simulink model "fangzhen"  (R2018a)
settings: Solver=FixedStepAuto  StartTime=0.0  StopTime=120  FixedStep=0.01  RelTol=1e-3
libraries: simulink x6
(part 1 of 2)
settings Model: Creator=WZJ  LastModifiedBy=Zijian
settings SolverCC: ZeroCrossAlgorithm=Adaptive
settings DebuggingCC: MaxConsecutiveZCsMsg=none

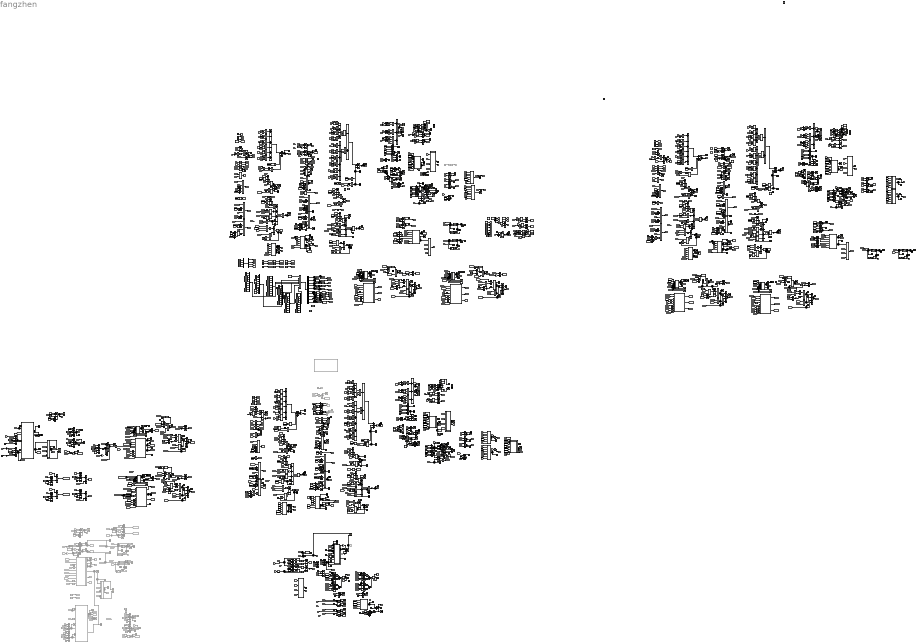
== system fangzhen ==
  note: 视野边界相撞
  note: 领导者机器人及其参数
  note: 相对坐标刚体队形
  note: 车辆模型
  note: 计算自变量
  note: 误差计算
  note: 切换初始位置k0
  note: 计算并选择过渡段,上界
  note: 误差模型1
  note: 控制器
  note: 选择过渡段
  note: theta i不等于theta id
  note: 控制器
  note: 计算接触斜率
  note: 角度界的计算
  note: 参数计算
  note: 计算过渡段
  note: 庄洁
  note: 后车角（此处theta和fai方向相反）
  note: 后车角误差
  note: 计算过渡段
  note: 计算自变量
  note: 误差模型1
  note: 后车角误差
  note: 选择过渡段
  note: 误差计算
  note: 控制器
  note: 角度界的计算
  note: 计算接触斜率
  note: theta i不等于theta id
  note: 计算接触斜率
  note: 选择过渡段
  note: 计算并选择过渡段,上界
  note: 控制器
  note: 庄洁
  note: 车辆模型
  note: 参数计算
  note: 切换初始位置k0
  note: 切换初始位置k0
  note: 计算过渡段
  note: 计算并选择过渡段,xia界
  note: 计算自变量
  note: 后车角（此处theta和fai方向相反）
  note: 误差计算
  note: theta i不等于theta id
  note: 参数计算
  note: 误差模型1
  note: 后车角（此处theta和fai方向相反）
  note: 控制器
  note: 控制器
  note: 车辆模型
  note: 庄洁
  note: 计算并选择过渡段,上界
  note: 计算并选择过渡段,xia界
  note: 计算自变量
  note: 计算接触斜率
  note: 计算过渡段
  note: 计算自变量
  note: 切换初始位置k0
  note: 计算接触斜率
  note: 后车角误差
  note: 选择过渡段
  note: 选择过渡段
  note: 切换初始位置k0
  note: 计算过渡段
  note: 选择过渡段
  note: 切换初始位置k0
  note: 计算接触斜率
  note: 计算过渡段
  note: 计算并选择过渡段,xia界
  note: 计算自变量
  note: 修正角（注意内部的正负）
  Abs{,1..5} (6 alike) : Abs
  Add{1,4,22,65,71,83,87,98..99,114,132..133,171,184,188,198..200} (18 alike) : Sum  Inputs=+--
  Add{10,13,15,17,21,23..24,28,34,36..40,43..46,50,52,55,59,62..63,69,73,76,85,95..96,101..102,104,106..107,109,113,115,117,120,122..123,129..130,134,136..139,143,147,149,153,160,162..163,166,168..169,173,176,186,195..196,225..227,233,236,240,263,267} (72 alike) : Sum  Inputs=+-
  Add{9,11..12,19,25,27,33,41,47,49,53,56..57,61,66,72,74,77..78,81,88..89,92,94,100,111,116,125,128,141,145,150,152,158,164,170,174,177..178,182,189..190,194,223,231,238,265,270} (48 alike) : Sum
  Add105 : Sum  Inputs=-+
  Add{2,16,35,51,108} (5 alike) : Sum  Inputs=+++
  Add{18,93,110,127,144,193,228,234} (8 alike) : Sum  Inputs=++-
  Add{20,112,146,175} (4 alike) : Sum  Inputs=+-+-
  Add{90..91,118,126,191..192} (6 alike) : Sum  Inputs=++--
  Add{119,135,140,224,230,264} (6 alike) : Sum  Inputs=++++
  Add{29,70,86,121,154,187} (6 alike) : Sum  Inputs=2
  Add{32,48,54,60,67..68,75,80,84,97,124,157,181,197} (14 alike) : Sum  Inputs=+-+
  Add14 : Sum  Inputs=-+
  Add{142,229,232,266} (4 alike) : Sum  Inputs=--
  Add148 : Sum  Inputs=+---
  Add{26,151,185,201,204..205,235,237,239} (9 alike) : Sum  Inputs=+-+--
  Add167 : Sum  Commented=on  Inputs=+--
  Add{172,207..208,210} (4 alike) : Sum  Commented=on  Inputs=+-+--
  Add{58,64,79,82,179,183} (6 alike) : Sum  Inputs=+++-
  Add180 : Sum  Commented=on  Inputs=+--
  Add211 : Sum  Commented=on  Inputs=+-+-
  Add212 : Sum  Commented=on  Inputs=+---
  Add213 : Sum  Commented=on  Inputs=+-+-
  Add214 : Sum  Commented=on  Inputs=+---
  Add42 : Sum  Inputs=-+
  Atan : Trigonometry  Operator=atan2
  Clock{2,5..6,8..11,24} (8 alike) : Clock
  Clock3 : Clock  Commented=on
  Clock4 : Clock  Commented=on
  Constant{1..3,49,54,56,69,72,79,98,118,124..125,138,147,161..162,175} (18 alike) : Constant  Value=3
  Constant{7,10,30,32,43,59,73,90,108,113,128,154,165..166,212,215,569..570,573} (19 alike) : Constant  Value=0.1
  Constant{8,23,25,28..29,31,33,35,46,48,53,64..66,70,74,84,87,91,94,100..102,109,111,117,123,134..135,140,145,151,156,160,171..172,177,192,213,264,289,293,543,564,568,572} (46 alike) : Constant
  Constant103 : Constant  Commented=on
  Constant{14,104..106,150,211,218} (7 alike) : Constant  Value=100
  Constant{4,62,85,93,107,132,157,169,214} (9 alike) : Constant  Value=0.01
  Constant{5,11,17,21..22,24,26..27,286..288} (11 alike) : Constant  Value=0.05
  Constant110 : Constant  Commented=on
  Constant{6,12..13,38..39,41,83,187,190,193..194} (11 alike) : Constant  Value=0
  Constant{18,50..51,57,67,82,89,95,120..121,126,149,153,155} (14 alike) : Constant  Value=pi*(87-7)/180
  Constant122 : Constant  Value=-0.3
  Constant127 : Constant  Value=1.5
  Constant{130,141,267,270,273,275,294,296,298} (9 alike) : Constant  Value=pi*87/180
  Constant133 : Constant  Value=0.2
  Constant{20,80..81,96..97,99,137,144,148,158..159,189,200..201,268..269,271,274,276,295,297,299,562} (23 alike) : Constant  Value=pi
  Constant143 : Constant  Value=pi*13/12
  Constant{9,15,78,86,92,565,567} (7 alike) : Constant  Value=10
  Constant152 : Constant  Value=0.3
  Constant{16,37,40,42} (4 alike) : Constant  Value=0.5
  Constant163 : Constant  Value=1.5
  Constant168 : Constant  Value=2
  Constant170 : Constant  Value=0.2
  Constant173 : Constant  Value=pi*13/12
  Constant{176,186,216,220} (4 alike) : Constant  Value=5
  Constant178 : Constant  Value=0.0001
  Constant182 : Constant  Value=50
  Constant185 : Constant  Value=20
  Constant19 : Constant  Value=-0.5
  Constant195 : Constant  Value=0.075
  Constant196 : Constant  Value=11.8  VectorParams1D=off
  Constant202 : Constant  Value=0.153  VectorParams1D=off
  Constant203 : Constant  Value=0.1  VectorParams1D=off
  Constant210 : Constant  Value=2
  Constant217 : Constant  Value=0.0001
  Constant219 : Constant  Value=20
  Constant243 : Constant  Value=-0.25
  Constant247 : Constant  Value=0.25
  Constant265 : Constant  Value=pi*11/12
  Constant36 : Constant  Value=6
  Constant{489,491,494,497,500,502} (6 alike) : Constant  Commented=on  Value=pi*87/180
  Constant490 : Constant  Commented=on  Value=-0.1
  Constant492 : Constant  Commented=on  Value=0.1
  Constant493 : Constant  Commented=on
  Constant{495..496,498,501,503} (5 alike) : Constant  Commented=on  Value=pi
  Constant499 : Constant  Commented=on  Value=-1
  Constant52 : Constant  Value=-0.3
  Constant{534,544,551,563} (4 alike) : Constant  Value=pi/2
  Constant538 : Constant  Value=1000
  Constant539 : Constant  Value=-0.5
  Constant545 : Constant  Value=pi*2
  Constant546 : Constant  Value=pi*3/2
  Constant547 : Constant  Commented=on  Value=pi/2
  Constant566 : Constant  Value=1000
  Constant63 : Constant  Value=0.2
  Constant68 : Constant  Value=0.15
  Constant71 : Constant  Value=0.15  VectorParams1D=off
  Constant75 : Constant  Commented=on  Value=2.828
  Constant76 : Constant  Commented=on  Value=pi*5/6
  Constant88 : Constant  Value=0.3
  Cos{1,3,7,11} (4 alike) : Trigonometry  Operator=cos
  Cos{2,4,8,12} (4 alike) : Trigonometry
  Demux : Demux  Outputs=10
  Demux1 : Demux
  Derivative{,1..45,47,50..58,61..64,66} (61 alike) : Derivative
  Divide{1..3,14..15,30,37,41,43,54..55,62} (12 alike) : Product
  Divide{5..6,9..11,21..22,25..27,35..36,38..40,42,45..46,49..51,60..61,63} (24 alike) : Product  Inputs=***
  Divide{7..8,12..13,23..24,28..29,47..48,52..53} (12 alike) : Product  Inputs=4
  Divide{16,18..19,31,33..34,56,58..59} (9 alike) : Product  Inputs=**
  Divide17 : Product  Inputs=3
  Divide20 : Product  Inputs=*/
  Divide32 : Product  Inputs=3
  Divide4 : Product  Inputs=*/
  Divide44 : Product  Inputs=*/
  Divide57 : Product  Inputs=3
  Foolower_1 : MATLAB Function  TreatAsAtomicUnit=on
  Foolower_2 : MATLAB Function  TreatAsAtomicUnit=on
  Foolower_3 : MATLAB Function  TreatAsAtomicUnit=on
  Foolower_4 : MATLAB Function  TreatAsAtomicUnit=on
  Foolower_5 : MATLAB Function  TreatAsAtomicUnit=on
  From1034 : From  Commented=on  GotoTag=xiajie_yuzhi_3
  From1046 : From  Commented=on  GotoTag=xi_pesai_3
  From1047 : From  Commented=on  GotoTag=xi_pesai_3_xia
  From{1087,1091,1093,1107..1108,1151} (6 alike) : From  Commented=on  GotoTag=pesai_d1_3
  From1088 : From  Commented=on  GotoTag=xi_pesai_0_xia_3
  From1089 : From  Commented=on  GotoTag=xi_shang
  From1090 : From  Commented=on  GotoTag=xi_xia
  From1092 : From  Commented=on  GotoTag=xi_pesai_0_3
  From1094 : From  Commented=on  GotoTag=pesai_d_a1_3
  From1095 : From  Commented=on  GotoTag=pesai_d_b1_3
  From{927,1097,1110,1148} (4 alike) : From  Commented=on  GotoTag=shang
  From{930,1098,1105,1113} (4 alike) : From  Commented=on  GotoTag=xia
  From1099 : From  Commented=on  GotoTag=xi_pesai_0_3
  From1100 : From  Commented=on  GotoTag=xi_pesai_0_xia_3
  From1101 : From  Commented=on  GotoTag=xi_pesai_0_3_qiehuan
  From1102 : From  Commented=on  GotoTag=xi_pesai_0_xia_3_qiehuan
  From1103 : From  Commented=on  GotoTag=xiajie_yuzhi_3
  From{1104,1109,1112,1147,1152} (5 alike) : From  Commented=on  GotoTag=fai_d_3
  From1106 : From  Commented=on  GotoTag=shangjie_yuzhi_3
  From1111 : From  Commented=on  GotoTag=pesai_d_3
  From1114 : From  Commented=on  GotoTag=pesai_d_3
  From1115 : From  Commented=on  GotoTag=pesai_d000
  From1118 : From  Commented=on  GotoTag=xi_shang
  From1119 : From  Commented=on  GotoTag=xi_xia
  From1143 : From  Commented=on  GotoTag=xi_pesai_3
  From1144 : From  Commented=on  GotoTag=xi_pesai_3_xia
  From1145 : From  Commented=on  GotoTag=shangjie_yuzhi_3
  From1146 : From  Commented=on  GotoTag=theta_id_3
  From1149 : From  Commented=on  GotoTag=ddd
  From1150 : From  Commented=on  GotoTag=theta_1
  From{934,1153..1155} (4 alike) : From  Commented=on  GotoTag=beta_3
  From932 : From  Commented=on  GotoTag=shang_
  From933 : From  Commented=on  GotoTag=xia_
  From935 : From  Commented=on  GotoTag=shangjie_yuzhi_3
  From938 : From  Commented=on  GotoTag=shang_
  From959 : From  Commented=on  GotoTag=xia_
  Gain{4,8..10,22..23,26,28,30,32,34,37,40,49,52,54,57,66,68..69,83..84,102} (23 alike) : Gain  Gain=-1
  Gain{13,24,41..44,71..72,75..76,100..101} (12 alike) : Gain  Gain=pi/2
  Gain{25,31,51,64..65,80,104,106..107} (9 alike) : Gain
  Gain{2..3,12,14..21,36,38..39,46..48,50} (18 alike) : Gain  Gain=0.5
  Gain{27,29,33,35,53,55} (6 alike) : Gain  Gain=3
  Gain{45,56,77..79} (5 alike) : Gain  Gain=-0.5
  Gain61 : Gain  Commented=on  Gain=-1
  Gain67 : Gain  Commented=on  Gain=-1
  Gain{81,86,91..92,95..96} (6 alike) : Gain  Commented=on  Gain=0.5
  Gain85 : Gain  Commented=on  Gain=-0.5
  Gain87 : Gain  Commented=on  Gain=-0.5
  Gain88 : Gain  Commented=on  Gain=-1
  Gain{89..90,93..94} (4 alike) : Gain  Commented=on
  Goto13 : Goto  Commented=on  GotoTag=l_d
  Goto19 : Goto  Commented=on  GotoTag=fai_d
  Goto243 : Goto  Commented=on  GotoTag=xi_pesai_3
  Goto263 : Goto  Commented=on  GotoTag=yipuxilong_pesai_3
  Goto290 : Goto  Commented=on  GotoTag=yipuxilong_pesai_3
  Goto325 : Goto  Commented=on  GotoTag=xi_pesai_3
  Goto368 : Goto  Commented=on  GotoTag=shang_
  Goto529 : Goto  Commented=on  GotoTag=xia_
  Goto534 : Goto  Commented=on  GotoTag=xi_pesai_0_xia_3_qiehuan
  Goto535 : Goto  Commented=on  GotoTag=xi_pesai_0_3_qiehuan
  Goto559 : Goto  Commented=on  GotoTag=yipuxilong_pesai_3
  Goto560 : Goto  Commented=on  GotoTag=pesai_d_b1_3
  Goto561 : Goto  Commented=on  GotoTag=pesai_d_a1_3
  Goto562 : Goto  Commented=on  GotoTag=beta_3
  Goto563 : Goto  Commented=on  GotoTag=xi_pesai_0_3
  Goto564 : Goto  Commented=on  GotoTag=xi_pesai_0_xia_3
  Goto565 : Goto  Commented=on  GotoTag=shangjie_yuzhi_3
  Goto566 : Goto  Commented=on  GotoTag=xiajie_yuzhi_3
  Goto567 : Goto  Commented=on  GotoTag=xi_pesai_3
  Goto568 : Goto  Commented=on  GotoTag=xi_pesai_3_xia
  Goto569 : Goto  Commented=on  GotoTag=ddd
  Goto570 : Goto  Commented=on  GotoTag=pesai_d_3
  Goto571 : Goto  Commented=on  GotoTag=pesai_d000
  Goto572 : Goto  Commented=on  GotoTag=xi_shang
  Goto573 : Goto  Commented=on  GotoTag=xi_xia
  Goto584 : Goto  Commented=on  GotoTag=C_3
  Integrator{5..8,10,15..18,20..22,24..29,34,39..44} (25 alike) : Integrator
  Integrator{9,11,30,45} (4 alike) : Integrator  InitialConditionSource=external
  Integrator12 : Integrator  InitialCondition=1.1
  Integrator13 : Integrator  InitialCondition=1
  Integrator14 : Integrator  InitialCondition=1.3
  Integrator19 : Integrator  InitialCondition=0.48236-0.1
  Integrator23 : Integrator  InitialCondition=-0.93185-0.5
  Integrator3 : Integrator  InitialCondition=0.8
  Integrator32 : Integrator  InitialCondition=0.8
  Integrator33 : Integrator  InitialCondition=-1
  Integrator35 : Integrator  InitialCondition=0.1
  Integrator36 : Integrator  InitialCondition=1.51763+0.1
  Integrator37 : Integrator  InitialCondition=-0.93185-0.5
  Integrator38 : Integrator  InitialCondition=1
  Integrator4 : Integrator  InitialCondition=0.1
  Integrator47 : Integrator  InitialCondition=-2.8637-0.5
  MATLAB Function : MATLAB Function  TreatAsAtomicUnit=on
  MATLAB Function1 : MATLAB Function  TreatAsAtomicUnit=on
  MATLAB Function10 : MATLAB Function  TreatAsAtomicUnit=on
  MATLAB Function13 : MATLAB Function  Commented=on  TreatAsAtomicUnit=on
  MATLAB Function14 : MATLAB Function  TreatAsAtomicUnit=on
  MATLAB Function15 : MATLAB Function  TreatAsAtomicUnit=on
  MATLAB Function16 : MATLAB Function  TreatAsAtomicUnit=on
  MATLAB Function17 : MATLAB Function  TreatAsAtomicUnit=on
  MATLAB Function2 : MATLAB Function  TreatAsAtomicUnit=on
  MATLAB Function20 : MATLAB Function  Commented=on  TreatAsAtomicUnit=on
  MATLAB Function22 : MATLAB Function  TreatAsAtomicUnit=on
  MATLAB Function23 : MATLAB Function  TreatAsAtomicUnit=on
  MATLAB Function25 : MATLAB Function  TreatAsAtomicUnit=on
  MATLAB Function26 : MATLAB Function  TreatAsAtomicUnit=on
  MATLAB Function27 : MATLAB Function  Commented=on  TreatAsAtomicUnit=on
  MATLAB Function29 : MATLAB Function  TreatAsAtomicUnit=on
  MATLAB Function3 : MATLAB Function  TreatAsAtomicUnit=on
  MATLAB Function30 : MATLAB Function  TreatAsAtomicUnit=on
  MATLAB Function32 : MATLAB Function  TreatAsAtomicUnit=on
  MATLAB Function36 : MATLAB Function  TreatAsAtomicUnit=on
  MATLAB Function37 : MATLAB Function  TreatAsAtomicUnit=on
  MATLAB Function38 : MATLAB Function  TreatAsAtomicUnit=on
  MATLAB Function39 : MATLAB Function  TreatAsAtomicUnit=on
  MATLAB Function4 : MATLAB Function  TreatAsAtomicUnit=on
  MATLAB Function47 : MATLAB Function  TreatAsAtomicUnit=on
  MATLAB Function48 : MATLAB Function  TreatAsAtomicUnit=on
  MATLAB Function49 : MATLAB Function  TreatAsAtomicUnit=on
  MATLAB Function50 : MATLAB Function  TreatAsAtomicUnit=on
  MATLAB Function52 : MATLAB Function  TreatAsAtomicUnit=on
  MATLAB Function7 : MATLAB Function  TreatAsAtomicUnit=on
  MATLAB Function8 : MATLAB Function  TreatAsAtomicUnit=on
  MATLAB 需要跑30s6 : MATLAB Function  TreatAsAtomicUnit=on
  Math Function{1..3,8..11,19..21,28,33,35,40..43,50} (18 alike) : Math  Operator=pow  SaturateOnIntegerOverflow=on
  Math Function{5..7,12..14,16..18,22..27,29..32,34,37..39,44..49,51} (30 alike) : Math  Operator=square  SaturateOnIntegerOverflow=on
  Math Function15 : Math  SaturateOnIntegerOverflow=on
  Math Function36 : Math  SaturateOnIntegerOverflow=on
  Math Function4 : Math  SaturateOnIntegerOverflow=on
  Memory{1..5,7..8,11..12,17,20..22,29..31,36..41} (22 alike) : Memory
  Memory{14..16,18..19,23..24} (7 alike) : Memory  Commented=on
  Multiport Switch : MultiPortSwitch
  Multiport Switch1 : MultiPortSwitch
  Multiport Switch2 : MultiPortSwitch
  Multiport Switch3 : MultiPortSwitch  Commented=on
  Multiport Switch4 : MultiPortSwitch  Inputs=6
  Mux{,1..3,6,15} (6 alike) : Mux  Inputs=10
  Mux7 : Mux
  Product{1,3,13..14,16,23,26,29..30,38,42,47,50,54,57,61,72,76,79..80,84..85,90..91,97,108,111..112,118,131,134,136,139,147,149,153,162,165..166,172..173,179} (42 alike) : Product  Inputs=**
  Product{5,10,12,17..18,21..22,24..25,28,33,37,39,45..46,52,56,58,62..63,65..66,74,82,87,89,94..95,98..100,103..107,109..110,113..116,119..125,127,130,133,138,140,144..145,148,150,154..155,157,160,168,170..171,180..184,186..195,197,202,205} (83 alike) : Product
  Product{19,32,34,40,101,141} (6 alike) : Product  Inputs=**/
  Product{20,48,51,59,71,75,102,151,161} (9 alike) : Product  Inputs=***/
  Product{6,11,27,35..36,43..44,55,64,67..68,73,77,126,128..129,132,142..143,156,158,163,196,198} (24 alike) : Product  Inputs=*/
  Product{96,117,178,185} (4 alike) : Product  Inputs=/*
  Product135 : Product  Commented=on  Inputs=/*
  Product137 : Product  Inputs=3
  Product{8,41,49,53,60,69..70,78,146,152,159,164} (12 alike) : Product  Inputs=**//
  Product15 : Product  Inputs=3
  Product167 : Product  Inputs=***
  Product169 : Product  Inputs=*/*
  Product31 : Product  Inputs=3
  Product81 : Product  Inputs=***
  Product83 : Product  Inputs=*/*
  Product86 : Product  Inputs=***
  Product88 : Product  Inputs=*/*
  Product93 : Product  Commented=on  Inputs=/*
  Saturation : Saturate  UpperLimit=0.04  LowerLimit=0
  Saturation Dynamic{,1..5} (6 alike) : simulink/Discontinuities/Saturation Dynamic  OutMin=[]  OutMax=[]  OutDataTypeStr=Inherit: Same as second input  OutDataType=fixdt(1, 16)  OutScaling=2^-10  DoSatur=off
  Saturation{1,3..4,9..11,16} (7 alike) : Saturate  UpperLimit=1  LowerLimit=-1
  Saturation12 : Saturate  UpperLimit=0.05  LowerLimit=0
  Saturation13 : Saturate  UpperLimit=0.05  LowerLimit=0
  Saturation{5,14..15,22..23,26} (6 alike) : Saturate  UpperLimit=0.1
  Saturation21 : Saturate  UpperLimit=0.05  LowerLimit=0
  Scope{1..30,32,34..35,37..40,42..48,50..80,82..84,86..88,90..115,117..127,129..135,137..166,168,170..173,175..201,203..219,221..222,224..228,230..236,238..242,244..245,247..248,250..257,259..265,267..269,271,273..282,284..286,290..297,299..301,306,310,312..316,318..320,322..323,325..328,339,345,347,349,368..371,378..387,389..393,401..404,408..420,423..424,428,469,472,475..476,478..486,490..495,504,506..508,514,516,518..519} (356 alike) : Scope
  Scope{36,41,81,85,89,116,167,169,202,220,223,266,270,283,289,311,321,324,348,421,427,488..489,505} (24 alike) : Scope  NumInputPorts=2
  Scope{31,49,128,229,388,405,477} (7 alike) : Scope  NumInputPorts=3
  Scope{237,243,246,336,350..353,358..362,364,367,372..376,422,426,430..436} (29 alike) : Scope  Commented=on
  Scope304 : Scope  Commented=on  NumInputPorts=3
  Scope{305,307..309,363,365..366,425,429} (9 alike) : Scope  Commented=on  NumInputPorts=2
  Sign : Signum
  Sign1 : Signum
  Sin{1,3,5..6,9..10} (6 alike) : Trigonometry  Operator=cos
  Square1 : Math  Operator=square  SaturateOnIntegerOverflow=on
  Square2 : Math  Operator=square  SaturateOnIntegerOverflow=on
  Square3 : Math  Operator=square  SaturateOnIntegerOverflow=on
  Subsystem1 : Subsystem
  Subsystem2 : Subsystem
  Subsystem3 : Subsystem
  Subsystem4 : Subsystem
  Subsystem5 : Subsystem
  Subtract1 : Sum  Inputs=++-
  Subtract{8..10,16,18,20,26..27,30,32,35,55..56,58..59,62..63,65..66} (19 alike) : Sum  Inputs=+-
  Subtract11 : Sum  Inputs=++-
  Subtract12 : Sum  Inputs=-+-+
  Subtract13 : Sum  Inputs=--+++-
  Subtract{4,14,24,31,33..34,36,60..61} (9 alike) : Sum  Inputs=-+
  Subtract15 : Sum  Inputs=++-+
  Subtract17 : Sum  Inputs=+-+-++
  Subtract{7,19,29,39..40,57,64,67..68} (9 alike) : Sum
  Subtract2 : Sum  Inputs=-+-+
  Subtract21 : Sum  Inputs=++-
  Subtract22 : Sum  Inputs=-+-+
  Subtract23 : Sum  Inputs=--+++-
  Subtract25 : Sum  Inputs=++-++
  Subtract28 : Sum  Inputs=+-+-++
  Subtract3 : Sum  Inputs=--+++-
  Subtract37 : Sum  Inputs=-++
  Subtract38 : Sum  Inputs=++-++
  Subtract5 : Sum  Inputs=+-+-++
  Subtract6 : Sum  Inputs=++-+
  Subtract71 : Sum  Inputs=+-+
  Subtract72 : Sum  Inputs=+-+
  Switch11 : Switch  Criteria=u2 > Threshold  Threshold=-0.5
  Switch12 : Switch  Criteria=u2 > Threshold  Threshold=0.5
  Switch{5,8..9,13} (4 alike) : Switch  Threshold=0.01
  Switch14 : Switch  Criteria=u2 > Threshold  Threshold=-0.5
  Switch17 : Switch  Commented=on  Criteria=u2 > Threshold  Threshold=0.1
  Switch18 : Switch  Commented=on  Threshold=0.00001
  Switch3 : Switch  Commented=on  Threshold=0.00001
  Switch4 : Switch  Commented=on  Criteria=u2 > Threshold  Threshold=-0.1
  Switch7 : Switch  Criteria=u2 > Threshold  Threshold=0.5
  To Workspace1 : ToWorkspace  VariableName=x0  SaveFormat=Structure  SampleTime=-1
  To Workspace11 : ToWorkspace  VariableName=x3  SaveFormat=Structure  SampleTime=-1
  To Workspace12 : ToWorkspace  VariableName=y3  SaveFormat=Structure  SampleTime=-1
  To Workspace2 : ToWorkspace  VariableName=y0  SaveFormat=Structure  SampleTime=-1
  To Workspace3 : ToWorkspace  VariableName=x2  SaveFormat=Structure  SampleTime=-1
  To Workspace6 : ToWorkspace  VariableName=x1  SaveFormat=Structure  SampleTime=-1
  To Workspace7 : ToWorkspace  VariableName=y1  SaveFormat=Structure  SampleTime=-1
  To Workspace8 : ToWorkspace  VariableName=y2  SaveFormat=Structure  SampleTime=-1
  Trigonometric Function{,1..2,5,8,11..12,15,18,24,26,28,30..34,36,42,44..49,51..52,55,58,61,67,69,71..74,82,89,94..96,98,100,103..104} (45 alike) : Trigonometry
  Trigonometric Function{3..4,6..7,9..10,13..14,16..17,19..23,25,27,29,35,37..41,43,50,53..54,56..57,59..60,62..66,68,87,90,92..93,97,99,105..106} (46 alike) : Trigonometry  Operator=cos
  Trigonometric Function88 : Trigonometry  Operator=atan2
  Trigonometric Function91 : Trigonometry  Operator=atan2
  tag scope: beta1=global
  wires:
  Constant264/1 -> [l_d_3], [l_d_2], [l_d]
  Product113/1 -> Add11/1
  Cos1/1 -> Product113/2
  [xL] -> Add11/2
  Product114/1 -> Add12/1
  Trigonometric Function29/1 -> Product116/1
  Constant265/1 -> [fai_d]
  Add11/1 -> [xLhead]
  [theta_L] -> Trigonometric Function29/1
  [theta_L] -> Cos1/1
  Integrator12/1 -> To Workspace2/1, [yL]  "yi"
  Integrator11/1 -> [theta_L]  "theta_i"
  [theta_L] -> Cos2/1
  Constant83/1 -> [oumiga_L_dot], [vL_dot]
  [theta_L] -> Trigonometric Function34/1
  Product115/1 -> Integrator12/1
  Cos2/1 -> Product114/2
  Constant143/1 -> [fai_d_2]
  Integrator13/1 -> To Workspace1/1, [xL]  "xi"
  Add102/1 -> [fai_d_3]
  Product116/1 -> Integrator13/1
  [oumiga_L] -> Integrator11/1
  [vL] -> Product116/2, Product115/1
  Trigonometric Function34/1 -> Product115/2
  [d] -> Product113/1
  Constant71/1 -> [h]
  [yL] -> Add12/2
  Add12/1 -> [yLhead]
  Constant68/1 -> [d]
  [d] -> Product114/1
  Add116/1 -> Scope250/1, [yF1head]
  [oumiga_1] -> Scope89/1
  Divide22/1 -> Subtract13/5
  Memory7/1 -> Switch13/1
  Constant2/1 -> Math Function1/2
  Constant20/1 -> Subtract15/4
  MATLAB Function/1(thetaid_0) -> Scope26/1, [theta_id_0]
  Math Function17/1 -> Product53/4
  Memory3/1 -> MATLAB Function2/6(d1b)
  [pesai_dot] -> Divide26/3
  Product72/1 -> Add80/2
  [u_21] -> Add86/1
  [pesai_d_b1] -> Multiport Switch/3
  Gain26/1 -> Scope113/1, [u_12]
  [pesai] -> Trigonometric Function13/1
  MATLAB Function3/1(V) -> [v1_dot_liju], Integrator6/1, Scope123/1
  Divide30/1 -> Subtract13/1
  Product103/1 -> Add108/1
  [h] -> MATLAB Function29/7(h)
  Divide26/1 -> Subtract5/3
  [e_pesai_dot] -> Product97/1
  Constant70/1 -> Add34/1
  [xi_pesai_0] -> MATLAB Function/1(x0)
  [vL] -> Divide38/1
  Constant62/1 -> [row_wuqiong]
  [yita_l] -> Add78/1
  [pesai_d1] -> Multiport Switch/4
  Add73/1 -> Product69/3
  Divide21/1 -> Subtract13/3
  Math Function16/1 -> Add125/2
  [pesai_d1] -> Scope49/1, MATLAB Function1/2(d1)
  Subtract11/1 -> Scope137/1, [gama_dot]
  [l] -> Divide20/2
  Math Function25/1 -> Add76/2
  Divide27/1 -> Subtract5/5
  [theta_id] -> MATLAB Function/3(thetaid)
  [yita_l] -> Product69/2
  [pesai_d1_00_a1] -> Memory3/1
  Saturation Dynamic/1 -> Product55/1
  Integrator6/1 -> [v1], Scope109/1
  Constant46/1 -> Add123/1
  [oumiga_id] -> Add97/3
  [fai] -> Trigonometric Function49/1
  [rou_0] -> Add122/1
  [xi_l] -> Product35/2
  [oumiga_1] -> Subtract16/2
  Saturation4/1 -> Product87/1
  Foolower_2/1(ldot) -> [l], Scope145/1
  [vL] -> MATLAB Function30/1(VL)
  [k_yita_pesai] -> Product8/1  "k_yita_pesai"
  Constant96/1 -> Add90/4
  [k_ke_xi_l] -> Product89/2  "k_ke_xi_l"
  Constant81/1 -> Add112/4
  [e_pesai_dot] -> Add83/1
  [xi_l] -> Product67/2
  Add81/1 -> Scope23/1, Product10/2
  Add37/1 -> Scope17/1, Product41/3
  [pesai] -> Trigonometric Function12/1
  [oumiga_L] -> Scope150/1, Add93/1
  Product37/1 -> Add88/2
  [fai] -> Trigonometric Function36/1
  [k_ke_xi_pesai] -> Product15/2  "k_ke_xi_pesai"
  Derivative28/1 -> [fai_dot], Scope85/2
  [oumiga_id] -> Add95/2
  [z_l] -> Math Function1/1
  Product11/1 -> Gain26/1
  Derivative36/1 -> [e_l_dot]
  Gain24/1 -> Add120/2
  [row_wuqiong] -> Add94/2
  Constant69/1 -> Math Function19/2
  [pesai_d1] -> Switch14/3
  Math Function19/1 -> Product89/1
  Subtract7/1 -> Scope120/1, [gama]
  [theta_L] -> Add1/2
  Product13/1 -> Scope155/1, Add82/1
  Clock10/1 -> Switch13/2
  Trigonometric Function37/1 -> Divide29/3
  [pesai_fin_a1] -> Scope16/1, Scope49/3, MATLAB Function1/4(fin)
  [c1_l] -> Product90/2
  [h] -> MATLAB Function30/7(h)
  [fai] -> Trigonometric Function39/1
  [yipuxilong_l_dot] -> Product71/1
  [theta_1] -> Add115/2
  [row_wuqiong] -> Add104/2
  [fai] -> Trigonometric Function37/1
  [k_tiaota_a1] -> Product107/1
  [yita_pesai] -> Math Function16/1
  Integrator18/1 -> [oumiga_1], Scope111/1
  [theta_L] -> Add67/2
  [v1] -> MATLAB Function29/2(Vi)
  Product47/1 -> Add83/2
  Gain2/1 -> Add1/3
  [e_pesai_dot] -> Add87/1
  Constant75/1 -> Goto13/1
  [z_l] -> Divide3/2
  Add113/1 -> Scope108/1
  [theta_id] -> Add67/1
  Product51/1 -> [c2_pesai]
  [shangjie_yuzhi] -> Add84/3
  [yLhead] -> Foolower_2/2(yl)
  [xi_pesai_x_a1] -> Product107/2
  Add99/1 -> Product84/1
  [fai_dot] -> Divide38/3
  Add100/1 -> [z_l]
  Divide24/1 -> Subtract13/6
  Derivative2/1 -> MATLAB Function2/4(d1_dotu)
  Gain15/1 -> Add84/2
  Product1/1 -> Add82/3
  [oumiga_L] -> MATLAB Function30/6(oumiga_L)
  Trigonometric Function12/1 -> Divide34/2
  [oumiga_1] -> Add97/2
  Divide29/1 -> Subtract5/6
  [shangjie_yuzhi] -> Add117/1
  [theta_1] -> Subsystem1/11(In11)
  MATLAB Function30/1(y) -> Scope381/1
  Add87/1 -> Product13/1
  [shangjie_yuzhi] -> MATLAB Function/6(shangjie_yuzhi)
  [shangjie_yuzhi] -> MATLAB Function2/2(shangjie_yuzhi)
  [pesai_d1] -> Derivative2/1
  [pesai_d1_dot_a1] -> Add120/1
  Add104/1 -> Product56/1
  Add123/1 -> Gain13/1
  [pesai] -> Trigonometric Function41/1
  [xF1head] -> Subsystem1/8(In8)
  Integrator14/1 -> [y1], To Workspace7/1  "yi"
  Product54/1 -> Add82/4
  [u_pesai_1] -> MATLAB Function3/6(u2)
  Add91/1 -> [pesai_d1], Scope87/1
  Switch13/1 -> Switch14/1
  [h] -> Divide35/1
  Add67/1 -> Scope70/1, [xi_pesai_0]
  MATLAB Function29/1(y) -> Scope380/1
  [oumiga_1] -> MATLAB Function29/5(oumiga_i)
  Integrator16/1 -> Subtract7/2
  [v1] -> MATLAB Function30/2(Vi)
  Product36/1 -> Scope161/1, [yita_pesai]
  [vL] -> MATLAB Function29/1(VL)
  Saturation5/1 -> Scope60/1
  [k_yita_pesai] -> Product41/1  "k_yita_pesai"
  [theta_id_0] -> Add75/1
  Add111/1 -> Scope257/1, [xF1head]
  [c_d_l] -> Product87/2  "自适应参数"
  Add117/1 -> Saturation Dynamic/2
  [l] -> MATLAB Function29/8(L)
  [k_c_l2] -> Product5/1  "k_c_l2"
  Add86/1 -> [u_l_1], Scope103/1
  [fai_dot] -> Divide29/4
  [xi_l] -> Derivative35/1
  Product41/1 -> Scope28/1, [ke_xi_pesai]
  [l_d] -> Product102/3
  [c1_pesai] -> Product34/1
  Trigonometric Function24/1 -> Product101/2
  [yita_l] -> Add50/2
  Gain13/1 -> Sin1/1
  [fai] -> MATLAB Function30/3(fai)
  Saturation3/1 -> Product33/1
  [pesai] -> MATLAB Function29/4(pesai)
  Product71/1 -> [c2_l]
  [rou_0] -> Gain24/1
  [ke_xi_l] -> Math Function18/1
  [theta_1] -> Subtract15/2
  [l] -> MATLAB Function3/3(l)
  [theta_L] -> Add91/1
  [oumiga_L] -> Add95/1
  [oumiga_L] -> Divide24/2
  [fai_d] -> Add110/1
  [d] -> Product101/3
  Product104/1 -> Add116/1
  [d] -> Product100/1
  [h] -> Divide24/1
  Gain21/1 -> Add114/3
  Add124/1 -> Gain22/1
  Subtract15/1 -> [fai], Scope71/1
  [oumiga_L_dot] -> Divide27/3
  Add112/1 -> Add105/1, Scope117/1
  Gain3/1 -> Add2/2
  Trigonometric Function25/1 -> Product102/2
  Constant63/1 -> [row_0]
  [yipuxilong_pesai] -> Add125/1
  Cos7/1 -> Product100/2
  [fai] -> MATLAB Function29/3(fai)
  [c3_l] -> Product91/1
  Math Function22/1 -> Add63/2
  Add96/1 -> [e_pesai], Scope92/1, Derivative1/1
  [pesai_d1_00_a1] -> Scope6/1, Add119/3
  [k_c_pesai] -> Product34/3  "k_c_pesai"
  [e_pesai] -> Product14/2
  Math Function26/1 -> Scope14/1, Product8/4
  [xi_pesai_0_xia] -> MATLAB Function/2(x0_xia)
  Switch5/1 -> Switch7/3
  [h] -> Divide29/1
  [c1_l] -> Divide3/1
  [xi_pesai_0] -> Scope53/1, Switch7/2
  [oumiga_L] -> Subtract11/2
  Math Function27/1 -> Product15/1
  Switch14/1 -> Scope68/1, Scope73/1, Memory7/1, Scope69/1
  [xiajie_yuzhi] -> Add2/3
  [oumiga_1] -> Add93/3, Scope165/1
  [pesai_d1_dot_a1] -> Memory5/1
  [pesai_d1] -> MATLAB Function2/5(d1_fnu)
  [pesai_d1] -> MATLAB Function2/3(d1u)
  MATLAB Function2/3(d1_fn) -> [pesai_fin_a1]
  [pesai_d_a1] -> Multiport Switch/2
  Multiport Switch/1 -> [pesai_d]
  [theta_L] -> Add2/1
  [oumiga_1] -> MATLAB Function30/5(oumiga_i)
  Product106/1 -> Scope4/1, Add119/1
  Constant57/1 -> Gain3/1
  [c1_pesai_dot] -> Product13/2
  Product6/1 -> [c3_pesai]
  Add83/1 -> Product42/1
  Add97/1 -> Scope38/1
  Product90/1 -> Scope10/1, Add100/1
  [k_ke_xi_l] -> Product86/2  "k_ke_xi_l"
  Product97/1 -> Add124/2, Scope115/1
  [oumiga_1] -> Divide35/3
  Product67/1 -> [yita_l]
  [e_l] -> Product91/2
  Product91/1 -> Add98/2
  [xLhead] -> Subsystem1/7(In7)
  [vL] -> Divide33/1
  Switch7/1 -> Scope45/1, Scope57/1, Memory11/1, Scope46/1
  [h] -> Divide28/1
  [v1] -> Divide34/1
  Gain27/1 -> Scope156/1, Add82/2
  Constant18/1 -> Gain20/1
  [yF1head] -> Subsystem1/5(In5)
  [fai_dot] -> Divide25/3
  Divide20/1 -> Scope132/1, Square2/1, [l_ni1]  "求逆"
  MATLAB Function1/2(a) -> Scope58/1
  [theta_1] -> Add107/2
  MATLAB Function/2(a) -> Scope7/1, Multiport Switch/1
  [oumiga_L] -> Divide29/2
  Cos8/1 -> Product104/2
  [xi_l] -> Product71/3
  [xi_pesai_0] -> MATLAB Function2/1(x0)
  Trigonometric Function44/1 -> Divide24/3
  [yita_pesai] -> Add81/1
  [c3_pesai] -> Product97/2
  Integrator8/1 -> [theta_id], Scope116/1, Scope42/1
  MATLAB Function2/1(d1) -> [pesai_d1_00_a1]
  Product33/1 -> Scope112/1, Add124/3
  [theta_L] -> Subtract15/3
  Gain14/1 -> Add67/3
  [k_c_pesai2] -> Product12/1
  Subtract13/1 -> Divide37/1
  [l_d] -> Subtract18/2
  Divide32/1 -> Subtract14/1
  [c2_pesai] -> Add87/3
  Derivative34/1 -> Scope157/1, [yipuxilong_pesai_dot]
  [e_pesai] -> Scope163/1, Product36/1
  Gain10/1 -> [u_21]
  [fai_d] -> Subtract8/2
  [l_ni2] -> Divide32/2
  [c3_l] -> Product72/2
  [h] -> Divide23/1
  [yipuxilong_l] -> Add77/1
  Product8/1 -> Scope160/1, [c1_pesai]
  [fai] -> Derivative28/1
  [oumiga_L] -> Product103/1
  Divide35/1 -> Subtract12/3
  [pesai] -> Subtract15/1
  Product89/1 -> Scope11/1, Add100/2
  [yita_pesai] -> Math Function22/1
  [pesai] -> MATLAB Function30/4(pesai)
  Add1/1 -> Scope25/1, [xi_pesai_0_xia]
  Add106/1 -> Trigonometric Function24/1
  [theta_L] -> Add75/2
  Constant97/1 -> Add91/4
  Add84/1 -> MATLAB Function/4(theta_shang_xiuzheng)
  Add88/1 -> [z_pesai]
  [ke_xi_pesai] -> Math Function27/1
  Constant50/1 -> Gain21/1
  [theta_1] -> Scope116/2
  [yipuxilong_l] -> Derivative17/1
  [e_pesai] -> Product47/2
  [theta_id_0] -> Add114/1
  Product98/1 -> Integrator14/1
  [yipuxilong_l] -> Add89/1
  [u_22] -> Add86/2
  [ke_xi_pesai_dot] -> Product15/3
  Math Function2/1 -> Scope8/1, Product1/2
  Derivative32/1 -> Scope51/1, [ke_xi_pesai_dot]
  [z_pesai] -> Divide1/2
  [c1_pesai] -> Derivative21/1
  Product73/1 -> Gain28/1
  Integrator27/1 -> Scope29/1
  Math Function15/1 -> Product56/2
  Derivative25/1 -> Scope85/1
  Add90/1 -> Scope169/2, Add96/1, Scope86/1
  [row_0] -> Add104/1
  [yipuxilong_pesai] -> Add81/2
  Math Function1/1 -> Scope9/1, Product3/2
  Divide31/1 -> Subtract5/1
  [v1] -> Product99/2, Product98/1
  [yita_pesai] -> Add37/2
  Integrator25/1 -> Math Function21/1, Scope20/1, [c_d_pesai]
  [xF1head] -> Subsystem1/3(In3)
  Product85/1 -> Add99/2
  [e_l_dot] -> Add99/1
  Product108/1 -> Scope15/1, Add79/4
  [theta_L] -> Add84/1
  Add77/1 -> Product71/4
  Divide23/1 -> Subtract13/4
  [xiajie_yuzhi] -> MATLAB Function/7(xiajie_yuzhi)
  Divide25/1 -> Subtract5/2
  Constant1/1 -> Math Function2/2
  Add50/1 -> Product66/1
  [e_l_dot] -> Product72/1
  [k_c_l] -> Product88/2  "k_c_l"
  Add49/1 -> Product41/4
  [theta_id] -> Add91/3
  [yita_pesai] -> Add49/1
  Product46/1 -> Math Function15/1
  [h] -> Divide27/1
  [yita_pesai] -> Product41/2
  Product100/1 -> Add111/1
  [h] -> MATLAB Function3/4(h)
  Subtract8/1 -> Scope83/1, Derivative25/1
  [theta_1] -> Add90/3
  Add23/1 -> Integrator25/1
  Subtract5/1 -> Add80/1
  [v1] -> Divide26/1
  [fai_dot] -> Divide24/4
  Divide28/1 -> Subtract5/4
  Memory11/1 -> Switch5/1
  [pesai_dot] -> Divide23/4
  Divide34/1 -> Subtract12/2
  Subtract12/1 -> Divide32/1
  [fai] -> Subtract7/1
  [yita_l] -> Add73/2
  [xi_pesai_x_a1] -> Product105/2
  Product56/1 -> Add94/1
  [u_12] -> Add121/2
  [c2_pesai] -> Add83/3
  Math Function24/1 -> Add89/2
  [theta_id] -> Add1/1
  [oumiga_1] -> Scope386/1, Integrator9/1
  [yF1head] -> Foolower_2/4(yf1head)
  Trigonometric Function38/1 -> Divide36/2
  [yita_l] -> Math Function24/1
  Add76/1 -> Product71/2
  Product88/1 -> Abs1/1
  Square2/1 -> [l_ni2], Scope126/1
  [yipuxilong_pesai] -> Scope18/1, Add66/1
  [yipuxilong_pesai_dot] -> Product51/1
  [e_l] -> Product85/2
  Divide3/1 -> Saturation4/1
  [k_yita_l] -> Product53/1  "k_yita_l"
  [c3_pesai] -> Product47/1
  Add121/1 -> [u_pesai_1], Scope65/1
  Product101/1 -> Add108/2
  Divide33/1 -> Subtract12/1
  MATLAB Function1/1(y) -> [pesai_d_a1], Derivative26/1, Scope47/1
  [theta_L] -> Add101/2
  [c1_l] -> Product88/3
  Product12/1 -> Add23/2
  Integrator15/1 -> [x1], To Workspace6/1  "xi"
  [vL_dot] -> Divide30/1
  [v1] -> Divide21/1
  [vL_dot] -> Divide31/1
  [pesai] -> Trigonometric Function42/1
  [fai_dot] -> Subtract11/1
  Gain29/1 -> Add79/2
  [yipuxilong_pesai] -> Derivative34/1
  Derivative35/1 -> [xi_l_dot]
  Product53/1 -> [c1_l]
  [ke_xi_pesai] -> Math Function28/1
  Math Function29/1 -> Add77/2
  Integrator9/1 -> Scope296/1, [theta_1]  "theta_i"
  [theta_1] -> Cos8/1
  [fai] -> Trigonometric Function40/1
  Sin1/1 -> Product106/2
  Gain28/1 -> Scope114/1, [u_22]
  [oumiga_1] -> Divide23/2
  [oumiga_1] -> Divide28/2
  Add85/1 -> Integrator26/1
  Trigonometric Function13/1 -> Divide35/2
  Product102/1 -> Add108/3
  [pesai_fin_a1] -> Memory8/1
  Add95/1 -> Add62/2, Integrator27/1
  Trigonometric Function35/1 -> Divide28/3
  Trigonometric Function41/1 -> Divide21/2
  [yita_l] -> Math Function25/1
  [z_l] -> Product108/1
  Product86/1 -> Gain29/1
  Product107/1 -> Scope5/1, Add119/2
  [c1_l] -> Derivative23/1
  [ke_xi_l_dot] -> ?
  Memory5/1 -> MATLAB Function2/7(d1_dotb)
  Constant48/1 -> Add37/1
  MATLAB Function3/2(W) -> Scope124/1, [oumiga_1_dot_liju], Integrator18/1
  [theta_1] -> Trigonometric Function14/1
  [c1_pesai] -> Product42/2
  Product14/1 -> Add87/2
  Add98/1 -> Product90/1
  [theta_id] -> Add112/2
  [xi_pesai] -> Scope162/1, Product36/2
  [gama] -> Add105/2
  [k_z_l] -> Product3/1
  [xi_pesai_dot] -> Product6/1
  [vL] -> Product101/1
  Integrator26/1 -> Math Function20/1, Scope80/1, [c_d_l]
  Constant54/1 -> Math Function20/2
  Add79/1 -> Product73/1
  [pesai] -> Scope169/1
  Trigonometric Function18/1 -> Product98/2
  Derivative30/1 -> [xi_pesai_dot]
  [theta_id] -> Add101/1
  [yipuxilong_l] -> Add74/2
  Gain22/1 -> [u_11], Scope24/1
  [pesai_dot] -> Divide21/3
  [e_l] -> Product67/1
  Add107/1 -> Scope144/1, [beta1]
  Constant76/1 -> Goto19/1
  [fai_d] -> Add112/3
  [e_l_dot] -> Add98/1
  [k_z_pesai] -> Product1/1
  Math Function21/1 -> Product12/2
  [z_pesai] -> Product54/1
  Add114/1 -> Product96/2, [xi_pesai_xia], Scope143/1
  [k_tiaota_a1] -> Product105/1
  [yita_l] -> Add76/1
  Math Function28/1 -> Product37/1
  Add80/1 -> Scope40/1, Gain10/1
  Add93/1 -> Add62/1, Scope166/1, Integrator5/1
  [theta_id] -> Add115/1
  [d] -> Product104/1
  [oumiga_L_dot] -> Divide22/3
  [xi_l_dot] -> Product35/1
  Integrator5/1 -> Scope43/1
  [xLhead] -> Subsystem1/2(In2)
  [rou_0] -> Product55/2
  [theta_L] -> Add114/2
  [xi_pesai] -> Derivative30/1
  [c1_l_dot] -> Product84/2
  Product69/1 -> [ke_xi_l]
  [k_ke_xi_pesai_dot] -> Product54/2
  [yita_l] -> Math Function29/1
  Product105/1 -> Add122/2
  MATLAB Function2/2(d1_dot) -> [pesai_d1_dot_a1]
  Divide1/1 -> Saturation3/1
  [theta_L] -> Add110/2
  Add119/1 -> [pesai_jie_a1], Scope48/1
  [xF1head] -> Foolower_2/3(xf1head)
  Add94/1 -> Scope110/1, Gain66/1, [xi_l]
  [pesai] -> Trigonometric Function35/1
  Product10/1 -> Math Function26/1
  Add62/1 -> Scope90/1
  Add2/1 -> MATLAB Function/5(theta_xia_xiuzheng)
  Divide38/1 -> Subtract13/2
  [x1] -> Add111/2
  [c3_l] -> Product85/1
  [oumiga_L] -> MATLAB Function29/6(oumiga_L)
  [theta_L] -> Add107/1
  Add89/1 -> Product53/2
  [theta_id] -> Add106/2
  Derivative17/1 -> [yipuxilong_l_dot]
  [pesai_jie_a1] -> Scope21/1, Scope49/2, MATLAB Function1/3(jie)
  Subtract14/1 -> Add124/1
  [c1_pesai] -> Divide1/1
  [ke_xi_l] -> Math Function19/1
  Derivative31/1 -> Scope32/1
  [fai] -> Add90/2
  [theta_L] -> Add112/1
  [d] -> Product102/4
  [theta_id] -> Add113/2
  Derivative23/1 -> [c1_l_dot]
  [u_11] -> Add121/1
  [oumiga_L] -> Product102/1
  [e_l] -> Derivative36/1
  [c2_l] -> Add99/3
  Derivative26/1 -> Saturation5/1
  [pesai_d1] -> Switch7/1
  [c2_l] -> Add98/3
  [y1] -> Add116/2
  Subtract18/1 -> Scope154/1, [e_l]
  Add120/1 -> [k_tiaota_a1]
  Trigonometric Function43/1 -> Divide22/2
  Constant49/1 -> Math Function28/2
  Trigonometric Function42/1 -> Divide23/3
  Constant59/1 -> [k_row]
  Add125/1 -> Product8/2
  [xi_pesai_x_a1] -> Add123/2
  [yita_l] -> Add74/1
  [xi_pesai] -> Product8/3
  [oumiga_1] -> Subtract11/3
  Trigonometric Function46/1 -> Divide30/2
  [h] -> Divide22/1
  Constant87/1 -> Divide20/1
  [xi_pesai_0] -> MATLAB Function1/1(x0)
  Gain4/1 -> Product46/2
  [ke_xi_pesai] -> Derivative32/1
  Divide36/1 -> Subtract12/4
  [fai_dot] -> Add93/2, Scope164/1
  [h] -> Divide36/1
  Trigonometric Function40/1 -> Divide38/2
  Trigonometric Function23/1 -> Product103/2
  Math Function23/1 -> Scope19/1, Add66/2
  [oumiga_L] -> Divide36/3
  [z_pesai] -> Math Function2/1
  [theta_1] -> Subsystem1/1(In1)
  Trigonometric Function19/1 -> MATLAB Function3/2(c)
  Add74/1 -> Product69/4
  [xi_pesai] -> Product51/3
  [k_ke_xi_pesai] -> Product37/2  "k_ke_xi_pesai"
  [pesai_dot] -> Divide28/4
  [c_d_pesai] -> Gain25/1  "自适应参数"
  [yLhead] -> Subsystem1/9(In9)
  [c3_pesai] -> Product14/1
  Gain20/1 -> Add75/3
  [fai] -> Trigonometric Function43/1
  [fai_d] -> Add91/2
  Add34/1 -> Scope22/1, Product10/1
  Constant53/1 -> Add73/1
  [theta_L] -> Add109/1
  [fai] -> Trigonometric Function38/1
  Add78/1 -> Product66/2
  [xLhead] -> Foolower_2/1(xl)
  Trigonometric Function39/1 -> Divide31/2
  Add101/1 -> Scope146/1
  Add66/1 -> Scope13/1, Product51/4
  [ke_xi_l] -> Derivative16/1
  [xi_pesai] -> Product6/2
  [fai] -> Trigonometric Function46/1
  Trigonometric Function49/1 -> Divide33/2
  [k_ke_xi_l_dot] -> Product108/2
  [theta_1] -> Trigonometric Function18/1
  [yita_pesai] -> Add34/2
  Trigonometric Function36/1 -> Divide27/2
  Product99/1 -> Integrator15/1
  Product55/1 -> Scope50/1, [xi_pesai_x_a1]
  Constant65/1 -> Add50/1
  Constant82/1 -> Gain14/1
  [l] -> Subtract18/1
  [fai_dot] -> Add97/1
  [yita_pesai] -> Add63/1
  Product42/1 -> Add88/1
  Add122/1 -> Product106/1
  [theta_1] -> Cos7/1
  [e_pesai] -> Derivative31/1
  Divide37/1 -> Subtract14/2
  [theta_id] -> Add110/3
  [xi_l] -> Product53/3
  [pesai] -> Trigonometric Function48/1
  Math Function18/1 -> Product86/1
  [xi_pesai_0_xia] -> Scope72/1, Switch14/2
  [z_l] -> Product88/1
  Add115/1 -> Scope119/1
  [pesai_d] -> Add96/2, Scope27/1
  [oumiga_L] -> Subtract16/1
  Trigonometric Function48/1 -> Divide26/2
  [theta_1] -> Subsystem1/6(In6)
  [yita_pesai] -> Math Function23/1
  [z_pesai] -> Product34/2
  Derivative1/1 -> [e_pesai_dot]
  Product3/1 -> Add79/3
  Constant64/1 -> [yipuxilong_l]
  Constant51/1 -> Gain2/1
  Add63/1 -> Product51/2
  Add109/1 -> Trigonometric Function23/1
  Subtract16/1 -> Integrator16/1
  Gain9/1 -> [yipuxilong_pesai], Scope147/1
  [theta_L] -> Add90/1
  [ke_xi_l_dot] -> Product86/3
  [yLhead] -> Subsystem1/4(In4)
  Add108/1 -> Scope89/2, [oumiga_id], Integrator8/1
  Constant56/1 -> Math Function21/2
  Add75/1 -> Product96/1, [xi_pesai], Scope125/1
  Product15/1 -> Gain27/1
  [pesai] -> Trigonometric Function19/1, Trigonometric Function11/1
  Add82/1 -> Product11/1
  [yF1head] -> Subsystem1/10(In10)
  Product35/1 -> [c3_l]
  Add105/1 -> Scope104/1
  Trigonometric Function47/1 -> Divide25/2
  Derivative21/1 -> [c1_pesai_dot]
  Constant89/1 -> Gain15/1
  [l_ni1] -> Divide37/2
  Memory8/1 -> MATLAB Function2/8(d1_fnb)
  [c1_pesai] -> Product11/2, Scope158/1
  Product66/1 -> Math Function17/1
  Clock2/1 -> Gain4/1
  [vL] -> Divide25/1
  Subsystem1/1(seita_i) -> Scope99/1
  Trigonometric Function14/1 -> Product99/1
  [theta_L] -> Add106/1
  Add110/1 -> Trigonometric Function25/1
  [yipuxilong_pesai] -> Add49/2
  Product96/1 -> Gain9/1
  Clock5/1 -> Switch5/2
  [k_yita_l] -> Product69/1  "k_yita_l"
  [fai] -> Subtract8/1
  [c1_l] -> Product73/2
  [theta_id] -> Add109/2
  Math Function20/1 -> Product5/2
  Product5/1 -> Add85/2
  Subsystem1/2(Out3) -> Scope159/1, Derivative33/1, [pesai]
  [theta_1] -> Add113/1
  [k_row] -> Product46/1
  [u_l_1] -> MATLAB Function3/5(u1)
  [fai] -> Trigonometric Function44/1
  Derivative16/1 -> [ke_xi_l_dot], Scope118/1
  [xi_pesai_0] -> Add117/2
  Trigonometric Function11/1 -> MATLAB Function3/1(s)
  [fai] -> Trigonometric Function47/1
  [l_dot] -> Divide32/3
  [yipuxilong_l] -> Add78/2
  Product84/1 -> Add79/1
  Product87/1 -> Add80/3
  [ke_xi_l_dot_2] -> ?
  [oumiga_L] -> Divide8/2
  [l_2] -> Divide4/2
  Product112/1 -> Add132/2
  [e_pesai_2] -> Scope141/1, Product44/1
  [d] -> Product19/3
  Trigonometric Function3/1 -> Divide39/2
  Add127/1 -> Add45/1, Scope153/1, Integrator22/1
  [yita_l_2] -> Add52/2
  [v2] -> Product120/2, Product119/1
  Gain43/1 -> Sin6/1
  [u_l_1_2] -> MATLAB Function10/5(u1)
  Constant28/1 -> Add143/1
  Divide10/1 -> Subtract17/3
  [xi_pesai_2] -> Product59/3
  [oumiga_2] -> Divide39/3
  [fai_2] -> Trigonometric Function15/1
  [pesai_d1_dot_a1_2] -> Add136/1
  Integrator20/1 -> Math Function10/1, Scope218/1, [c_d_l_2]
  Derivative13/1 -> Scope220/1
  Add71/1 -> Product29/1
  Cos3/1 -> Product18/2
  Product50/1 -> Add72/1
  MATLAB Function10/1(V) -> [v2_dot_liju], Integrator28/1, Scope94/1
  Subtract6/1 -> [fai_2], Scope214/1
  [e_l_dot_2] -> Product76/1
  [fai_dot_2] -> Divide9/3
  Derivative22/1 -> [xi_pesai_dot_2]
  Trigonometric Function16/1 -> Divide13/3
  Divide42/1 -> Subtract3/2
  Product81/1 -> Gain35/1
  Add46/1 -> Product59/2
  [xi_pesai_0_xia_2] -> Scope215/1, Switch11/2
  Product17/1 -> Math Function31/1
  Add126/1 -> [pesai_d1_2], Scope222/1
  [h] -> Divide6/1
  MATLAB Function7/1(thetaid_0) -> Scope179/1, [theta_id_0_2]
  [theta_L] -> Add54/2
  Gain36/1 -> Add35/2
  [pesai_dot_2] -> Divide10/3
  [u_22_2] -> Add70/2
  Derivative41/1 -> [xi_l_dot_2]
  [yita_pesai_2] -> Product49/2
  [yipuxilong_l_2] -> Add53/2
  Add55/1 -> Product75/2
  Trigonometric Function4/1 -> Product120/1
  [oumiga_2] -> Subtract1/3
  Add129/1 -> Add45/2, Integrator21/1
  Product26/1 -> Scope122/1, Add58/4
  Subsystem2/1(seita_i) -> Scope227/1
  [theta_2] -> Add118/3
  [h] -> MATLAB Function25/7(h)
  [xi_pesai_2] -> Product64/2
  [pesai_2] -> Trigonometric Function10/1
  [oumiga_2] -> Subtract9/2
  Math Function9/1 -> Scope217/1, Product16/2
  Add56/1 -> Product75/4
  [theta_id_2] -> Add48/1
  [h] -> MATLAB Function26/7(h)
  Math Function34/1 -> Add56/2
  [e_pesai_2] -> Product30/2
  Integrator10/1 -> [oumiga_2], Scope75/1
  [v2] -> MATLAB Function26/2(Vi)
  [c_d_l_2] -> Product82/2  "自适应参数"
  Add35/1 -> MATLAB Function7/5(theta_xia_xiuzheng)
  Math Function5/1 -> Add33/2
  [pesai_d1_2] -> MATLAB Function17/3(d1u)
  Divide9/1 -> Subtract17/2
  Constant151/1 -> Divide4/1
  Multiport Switch1/1 -> [pesai_d_2]
  [c1_l_2] -> Product83/3
  Derivative11/1 -> [c1_l_dot_2]
  [xiajie_yuzhi_2] -> MATLAB Function7/7(xiajie_yuzhi)
  [theta_id_0_2] -> Add22/1
  Derivative44/1 -> MATLAB Function17/4(d1_dotu)
  [shangjie_yuzhi_2] -> MATLAB Function15/2(shangjie_yuzhi)
  Product117/1 -> Gain40/1
  Gain41/1 -> Sin5/1
  Product19/1 -> Add16/2
  [pesai_2] -> Trigonometric Function26/1
  Trigonometric Function30/1 -> Divide15/2
  [oumiga_2] -> MATLAB Function25/5(oumiga_i)
  Divide16/1 -> Subtract17/1
  [yita_pesai_2] -> Add41/1
  Constant125/1 -> Math Function11/2
  [fai_dot_2] -> Divide13/4
  [e_pesai_2] -> Derivative37/1
  Trigonometric Function6/1 -> MATLAB Function10/2(c)
  [theta_L] -> Add4/2
  Switch12/1 -> Scope59/1, Scope185/1, Memory12/1, Scope172/1
  Gain23/1 -> [u_11_2], Scope177/1
  [vL_dot] -> Divide16/1
  Clock11/1 -> Gain37/1
  [theta_2] -> Add24/2
  Derivative5/1 -> [e_pesai_dot_2]
  [oumiga_L] -> Scope127/1, Add127/1
  [oumiga_L] -> MATLAB Function25/6(oumiga_L)
  Add33/1 -> Product78/2
  [h] -> Divide13/1
  [c3_l_2] -> Product80/1
  [pesai_d1_dot_b1_2] -> Add141/1
  [yipuxilong_pesai_2] -> Scope170/1, Add47/1
  [yipuxilong_pesai_dot_2] -> Product59/1
  MATLAB Function17/2(d1_dot) -> [pesai_d1_dot_b1_2]
  Clock9/1 -> Switch9/2
  [c2_l_2] -> Add132/3
  Math Function30/1 -> Add55/2
  Divide4/1 -> Scope100/1, Square1/1, [l_ni1_2]  "求逆"
  Divide7/1 -> Subtract3/4
  MATLAB Function15/3(d1_fn) -> [pesai_fin_a1_2]
  Constant148/1 -> Add20/4
  Trigonometric Function31/1 -> Divide9/2
  [pesai_2] -> MATLAB Function25/4(pesai)
  [vL_dot] -> Divide15/1
  [u_pesai_1_2] -> MATLAB Function10/6(u2)
  Subsystem2/2(Out3) -> Scope135/1, [pesai_2]
  Trigonometric Function9/1 -> Product20/2
  Add92/1 -> Product60/2
  [yipuxilong_l_2] -> Add56/1
  Memory20/1 -> MATLAB Function17/6(d1b)
  [fai_2] -> MATLAB Function25/3(fai)
  [theta_id_2] -> Add10/1
  Clock8/1 -> Switch8/2
  [c_d_pesai_2] -> Gain31/1  "自适应参数"
  Product22/1 -> Add25/1
  [xi_pesai_2] -> Derivative22/1
  Add118/1 -> Scope167/2, Add130/1, Scope221/1
  Trigonometric Function17/1 -> Divide40/2
  [z_pesai_2] -> Product40/2
  Saturation14/1 -> Scope149/1
  [xi_pesai_x_b1_2] -> Product124/2
  Memory2/1 -> MATLAB Function15/6(d1b)
  Add58/1 -> Product77/1
  [theta_L] -> Add20/1
  Derivative18/1 -> [fai_dot_2], Scope220/2
  [fai_2] -> Trigonometric Function30/1
  [c1_pesai_2] -> Derivative10/1
  [xi_pesai_0_2] -> Add134/2
  [k_c_l_2] -> Product83/2  "k_c_l"
  Add19/1 -> [xF2head]
  Constant121/1 -> Gain17/1
  [theta_L] -> Add15/1
  [v2] -> Divide19/1
  Cos4/1 -> Product22/2
  Math Function14/1 -> Add92/2
  [pesai_jie_b1_2] -> Scope31/2, MATLAB Function16/3(jie)
  [e_pesai_dot_2] -> Product118/1
  Add136/1 -> [k_tiaota_a1_2]
  [yita_pesai_2] -> Add39/2
  Constant135/1 -> Add43/1
  Divide40/1 -> Subtract2/4
  [v2] -> MATLAB Function25/2(Vi)
  [pesai_2] -> MATLAB Function26/4(pesai)
  MATLAB Function26/1(y) -> Scope277/1
  [l_2] -> MATLAB Function25/8(L)
  [vL] -> MATLAB Function25/1(VL)
  Product29/1 -> Scope130/1, Add64/1
  Add138/1 -> Gain41/1
  Product109/1 -> Scope67/1, Add9/2
  [pesai_d1_dot_a1_2] -> Memory4/1
  [xi_pesai_x_a1_2] -> Add138/2
  Memory21/1 -> MATLAB Function15/8(d1_fnb)
  Memory22/1 -> MATLAB Function17/7(d1_dotb)
  [k_z_pesai_2] -> Product16/1
  [pesai_d1_00_b1_2] -> Memory20/1
  Gain32/1 -> Scope77/1, [u_12_2]
  Math Function3/1 -> Scope224/1, Product38/2
  [pesai_d1_2] -> Scope229/1, MATLAB Function4/2(d1)
  [xi_pesai_0_xia_2] -> MATLAB Function7/2(x0_xia)
  MATLAB Function16/1(y) -> [pesai_d_b1_2], Derivative45/1, Scope2/1
  [k_tiaota_b1_2] -> Product124/1
  [xi_pesai_0_xia_2] -> MATLAB Function16/1(x0)
  [pesai_d1_2] -> MATLAB Function15/3(d1u)
  MATLAB Function15/1(d1) -> [pesai_d1_00_a1_2]
  Constant98/1 -> Math Function3/2
  [pesai_dot_2] -> Divide12/4
  [theta_L] -> Add22/2
  [pesai_fin_a1_2] -> Memory21/1
  [pesai_d1_2] -> Derivative44/1
  Gain42/1 -> Add136/2
  Add135/1 -> [pesai_jie_a1_2], Scope228/1
  [shangjie_yuzhi_2] -> Add134/1
  [fai_d_2] -> Add18/1
  [yipuxilong_pesai_2] -> Derivative40/1
  [xi_l_2] -> Product43/2
  [vL] -> Product19/1
  [k_tiaota_a1_2] -> Product123/1
  [pesai_d1_00_b1_2] -> Scope148/1, Add140/3
  Divide2/1 -> Saturation9/1
  Product39/1 -> Scope76/1, Add32/3
  [ke_xi_pesai_2] -> Math Function32/1
  [theta_L] -> Add118/1
  [theta_id_2] -> Add24/1
  Gain12/1 -> Add48/3
  [pesai_fin_b1_2] -> Memory1/1
  [theta_L] -> Add48/2
  Add45/1 -> Scope225/1
  [yita_pesai_2] -> Add40/2
  Constant140/1 -> Add39/1
  Product119/1 -> Integrator3/1
  [c3_l_2] -> Product76/2
  [pesai_dot_2] -> Divide7/4
  Divide41/1 -> Subtract4/2
  Constant124/1 -> Math Function10/2
  Trigonometric Function33/1 -> Divide18/2
  [oumiga_L] -> Subtract1/2
  [pesai_2] -> Trigonometric Function3/1
  [yita_pesai_2] -> Math Function13/1
  Constant120/1 -> Gain19/1
  [fai_2] -> Trigonometric Function28/1
  [oumiga_2] -> Divide7/2
  [yF2head] -> Foolower_1/4(yf1head)
  [row_wuqiong_2] -> Add128/2
  Divide15/1 -> Subtract3/1
  Math Function33/1 -> Product45/1
  Subtract4/1 -> Add32/1
  [theta_2] -> Subsystem2/11(In11)
  Product58/1 -> Add69/2
  Math Function31/1 -> Scope102/1, Product78/4
  Constant123/1 -> Add52/1
  [oumiga_id_2] -> Add129/2
  Subtract17/1 -> Add60/1
  [oumiga_L_dot] -> Divide6/3
  Trigonometric Function28/1 -> Divide8/3
  Add43/1 -> Product65/1
  Product59/1 -> [c2_pesai_2]
  [theta_L] -> Add10/2
  Product76/1 -> Add60/2
  Add21/1 -> Scope64/1
  Saturation15/1 -> Scope234/1
  [d] -> Product18/1
  [fai_d_2] -> Add126/2
  Trigonometric Function27/1 -> Divide6/2
  [k_c_pesai_2] -> Product40/3  "k_c_pesai"
  [row_0_2] -> Add13/1
  Product118/1 -> Add32/2, Scope79/1
  [theta_2] -> Trigonometric Function5/1
  [xi_pesai_x_a1_2] -> Product121/2
  [oumiga_L] -> Subtract9/1
  [xi_pesai_x_b1_2] -> Add143/2
  MATLAB Function10/2(W) -> Scope95/1, [oumiga_2_dot_liju], Integrator10/1
  [pesai_d1_2] -> Derivative27/1
  Constant138/1 -> Math Function8/2
  [z_pesai_2] -> Divide2/2
  Add133/1 -> Product79/1
  Constant158/1 -> Add118/4
  Product63/1 -> Add128/1
  Add24/1 -> Scope88/1
  [c1_pesai_2] -> Product40/1
  Subtract9/1 -> Integrator7/1
  [fai_dot_2] -> Subtract1/1
  Product52/1 -> Math Function4/1
  [xLhead] -> Subsystem2/2(In2)
  [yLhead] -> Foolower_1/2(yl)
  Divide17/1 -> Subtract4/1
  [e_pesai_dot_2] -> Add65/1
  [yita_l_2] -> Add43/2
  [u_12_2] -> Add29/2
  [fai_dot_2] -> Divide42/3
  Trigonometric Function22/1 -> Divide5/2
  [z_l_2] -> Math Function3/1
  [vL] -> MATLAB Function26/1(VL)
  Add60/1 -> Scope195/1, Gain8/1
  Math Function4/1 -> Product63/2
  [k_c_pesai2_2] -> Product28/1
  [oumiga_L] -> Divide13/2
  [xi_pesai_0_2] -> MATLAB Function7/1(x0)
  [c1_pesai_dot_2] -> Product29/2
  Add69/1 -> Integrator20/1
  [theta_id_2] -> Add15/2
  Divide18/1 -> Subtract2/1
  [pesai_dot_2] -> Divide5/3
  Product123/1 -> Scope230/1, Add135/2
  [pesai_2] -> Trigonometric Function2/1
  Constant23/1 -> Add138/1
  [v2] -> Divide5/1
  [c1_pesai_2] -> Product50/2
  [fai_2] -> Trigonometric Function21/1
  Trigonometric Function32/1 -> Divide10/2
  [oumiga_L] -> Product21/1
  Divide14/1 -> Saturation10/1
  Math Function6/1 -> Product60/4
  [z_l_2] -> Divide14/2
  Constant126/1 -> Gain36/1
  Divide12/1 -> Subtract17/4
  [pesai_d_a1_2] -> Multiport Switch1/2
  [yipuxilong_pesai_2] -> Add33/1
  [fai_2] -> MATLAB Function26/3(fai)
  [v2] -> Divide10/1
  Gain17/1 -> Add4/3
  [xi_l_2] -> Product75/3
  [pesai_2] -> Trigonometric Function6/1, Trigonometric Function1/1
  [l_d_2] -> Product20/3
  Math Function32/1 -> Product31/1
  [ke_xi_l_2] -> Math Function8/1
  Add10/1 -> Scope107/1
  [xF2head] -> Foolower_1/3(xf1head)
  [pesai_2] -> Scope167/1
  Product83/1 -> Abs2/1
  Product44/1 -> Scope139/1, [yita_pesai_2]
  Derivative38/1 -> Scope205/1, [ke_xi_pesai_dot_2]
  Product68/1 -> [yita_l_2]
  [l_2] -> Subtract10/1
  [fai_dot_2] -> Divide8/4
  Product60/1 -> [c1_l_2]
  Add130/1 -> [e_pesai_2], Scope226/1, Derivative5/1
  Gain35/1 -> Add58/2
  Integrator28/1 -> [v2], Scope66/1
  [theta_id_2] -> Add17/2
  Saturation10/1 -> Product82/1
  [c3_pesai_2] -> Product118/2
  Add128/1 -> Scope74/1, Gain68/1, [xi_l_2]
  Product43/1 -> [c3_l_2]
  [c3_pesai_2] -> Product57/1
  [e_l_2] -> Derivative42/1
  [yLhead] -> Subsystem2/4(In4)
  Product126/1 -> Scope231/1, [xi_pesai_x_a1_2]
  Divide19/1 -> Subtract2/2
  Divide39/1 -> Subtract2/3
  Product111/1 -> Scope61/1, Add9/1
  [theta_L] -> Add126/1
  [fai_2] -> Trigonometric Function33/1
  Add61/1 -> Scope176/1, Product17/2
  [yita_l_2] -> Product70/2
  Add29/1 -> [u_pesai_1_2], Scope209/1
  [xiajie_yuzhi_2] -> Add35/3
  [k_z_l_2] -> Product38/1
  [k_ke_xi_pesai_2] -> Product45/2  "k_ke_xi_pesai"
  Add64/1 -> Product27/1
  [pesai_d_b1_2] -> Multiport Switch1/3
  Constant117/1 -> Add40/1
  [xi_pesai_0_2] -> Scope183/1, Switch12/2
  [pesai_fin_a1_2] -> Scope229/3, MATLAB Function4/4(fin)
  Trigonometric Function2/1 -> Divide19/2
  Add65/1 -> Product50/1
  Add72/1 -> [z_pesai_2]
  [theta_L] -> Add35/1
  [d] -> Product22/1
  Integrator22/1 -> Scope198/1
  [fai_2] -> Add118/2
  [yita_pesai_2] -> Math Function12/1
  [theta_id_2] -> Add21/2
  Product64/1 -> [c3_pesai_2]
  Product30/1 -> Add71/2
  [xLhead] -> Foolower_1/1(xl)
  Product78/1 -> Scope138/1, [c1_pesai_2]
  [fai_2] -> Trigonometric Function17/1
  Add141/1 -> [k_tiaota_b1_2]
  Gain33/1 -> Scope131/1, Add64/2
  Product20/1 -> Add16/3
  [theta_2] -> Cos4/1
  Derivative37/1 -> Scope186/1
  [d] -> Product20/4
  Product77/1 -> Gain34/1
  Constant149/1 -> Gain12/1
  [xLhead] -> Subsystem2/7(In7)
  [xi_pesai_2] -> Scope140/1, Product44/2
  Add53/1 -> Product70/4
  [pesai_d1_2] -> Multiport Switch1/4
  Subtract1/1 -> Scope101/1
  [oumiga_2] -> Scope223/1
  [yipuxilong_l_2] -> Add92/1
  Integrator29/1 -> [theta_id_2], Scope81/1, Scope197/1
  Constant159/1 -> Add126/4
  [yF2head] -> Subsystem2/5(In5)
  Memory1/1 -> MATLAB Function17/8(d1_fnb)
  Divide11/1 -> Subtract17/5
  Trigonometric Function5/1 -> Product119/2
  [k_tiaota_b1_2] -> Product127/1
  [theta_2] -> Trigonometric Function4/1
  Add22/1 -> Product117/2, [xi_pesai_2_xia], Scope105/1
  [pesai_d1_dot_b1_2] -> Memory22/1
  [theta_id_2] -> MATLAB Function7/3(thetaid)
  [theta_2] -> Cos3/1
  Switch9/1 -> Switch11/1
  Product45/1 -> Add72/2
  Foolower_1/1(ldot) -> [l_2], Scope106/1
  [h] -> Divide39/1
  Math Function8/1 -> Product109/1
  Saturation9/1 -> Product39/1
  [vL] -> Divide9/1
  [theta_2] -> Subsystem2/1(In1)
  [c1_l_2] -> Derivative11/1
  Integrator7/1 -> Subtract19/2
  Add25/1 -> [yF2head]
  [c1_l_2] -> Product111/2
  [k_ke_xi_pesai_2] -> Product31/2  "k_ke_xi_pesai"
  Add52/1 -> Product70/3
  [z_l_2] -> Product83/1
  Product121/1 -> Add137/2
  [gama_2] -> Add14/2
  Product79/1 -> Add58/1
  Gain40/1 -> [yipuxilong_pesai_2], Scope121/1
  [ke_xi_l_2] -> Math Function7/1
  [yita_l_2] -> Add55/1
  Derivative42/1 -> [e_l_dot_2]
  [xi_pesai_0_xia_2] -> Add139/1
  Derivative6/1 -> [ke_xi_l_dot_2], Scope84/1
  Add68/1 -> MATLAB Function7/4(theta_shang_xiuzheng)
  [c1_l_2] -> Product77/2
  Subtract2/1 -> Divide17/1
  Product38/1 -> Add58/3
  MATLAB Function25/1(y) -> Scope276/1
  [yipuxilong_l_2] -> Add57/2
  [e_l_2] -> Product80/2
  Add17/1 -> Trigonometric Function7/1
  Add140/1 -> [pesai_jie_b1_2], Scope3/1
  [pesai_d1_2] -> Scope31/1, MATLAB Function16/2(d1)
  [h] -> Divide8/1
  Derivative40/1 -> Scope133/1, [yipuxilong_pesai_dot_2]
  Add32/1 -> Gain23/1
  [fai_2] -> Trigonometric Function20/1
  [e_l_dot_2] -> Add132/1
  [xF2head] -> Subsystem2/3(In3)
  Gain19/1 -> Add22/3
  [xi_pesai_2] -> Product78/3
  [fai_2] -> Derivative18/1
  [xi_l_2] -> Product68/2
  [h] -> Divide12/1
  [pesai_d1_2] -> MATLAB Function15/5(d1_fnu)
  [oumiga_2] -> MATLAB Function26/5(oumiga_i)
  [xi_pesai_x_a1_2] -> Product123/2
  [yF2head] -> Subsystem2/10(In10)
  Product28/1 -> Add36/2
  [yita_l_2] -> Math Function30/1
  [theta_2] -> Subtract6/2
  Add39/1 -> Scope175/1, Product17/1
  [yita_l_2] -> Add57/1
  Add47/1 -> Scope98/1, Product59/4
  [oumiga_L] -> MATLAB Function26/6(oumiga_L)
  [oumiga_2] -> Divide12/2
  [h] -> Divide40/1
  [z_pesai_2] -> Math Function9/1
  MATLAB Function4/1(y) -> [pesai_d_a1_2], Derivative29/1, Scope152/1
  Add137/1 -> Product122/1
  Gain37/1 -> Product52/2
  Constant128/1 -> [k_row_2]
  [xi_l_dot_2] -> Product43/1
  [c3_pesai_2] -> Product30/1
  Trigonometric Function21/1 -> Divide42/2
  Sin6/1 -> Product125/2
  [fai_2] -> Subtract19/1
  [c1_l_2] -> Divide14/1
  Product128/1 -> Scope54/1, [xi_pesai_x_b1_2]
  [fai_2] -> Trigonometric Function27/1
  [yipuxilong_l_dot_2] -> Product75/1
  [pesai_fin_b1_2] -> Scope31/3, MATLAB Function16/4(fin)
  [rou_0_2] -> Gain42/1, Add137/1, Product126/2
  [theta_id_0_2] -> Add54/1
  [oumiga_2] -> Scope385/1, Integrator30/1
  [u_21_2] -> Add70/1
  Divide5/1 -> Subtract3/3
  Product16/1 -> Add64/3
  [theta_id_2] -> Add20/2
  [c1_l_dot_2] -> Product79/2
  Trigonometric Function15/1 -> Divide11/2
  Add14/1 -> Scope63/1
  [e_pesai_dot_2] -> Add71/1
  Product127/1 -> Scope52/1, Add140/2
  Constant132/1 -> [row_wuqiong_2]
  [k_tiaota_a1_2] -> Product121/1
  Add15/1 -> Trigonometric Function8/1
  [oumiga_L] -> Divide40/3
  Add9/1 -> [z_l_2]
  Add20/1 -> Add14/1, Scope82/1
  [fai_dot_2] -> Add127/2, Scope142/1
  [theta_L] -> Add18/2
  [k_yita_l_2] -> Product70/1  "k_yita_l"
  [l_d_2] -> Subtract10/2
  Constant133/1 -> [row_0_2]
  [k_yita_l_2] -> Product60/1  "k_yita_l"
  [theta_id_2] -> Add4/1
  Subtract20/1 -> Scope219/1, Derivative13/1
  [k_yita_pesai_2] -> Product49/1  "k_yita_pesai"
  [h] -> Divide7/1
  [pesai_d1_2] -> MATLAB Function17/5(d1_fnu)
  [pesai_d1_00_a1_2] -> Memory2/1
  [pesai_d_2] -> Add130/2, Scope180/1
  [yipuxilong_pesai_2] -> Add41/2
  Gain34/1 -> Scope78/1, [u_22_2]
  Add142/1 -> Product125/1
  [ke_xi_pesai_2] -> Math Function33/1
  [vL] -> Divide18/1
  [k_ke_xi_pesai_dot_2] -> Product61/2
  Product40/1 -> Abs3/1
  Derivative10/1 -> [c1_pesai_dot_2]
  Derivative27/1 -> MATLAB Function15/4(d1_dotu)
  Constant134/1 -> [yipuxilong_l_2]
  Add143/1 -> Gain43/1
  [yLhead] -> Subsystem2/9(In9)
  Add132/1 -> Product111/1
  Memory17/1 -> Switch9/1
  Constant118/1 -> Math Function33/2
  [yita_pesai_2] -> Add46/1
  [yita_pesai_2] -> Math Function5/1
  [ke_xi_pesai_dot_2] -> Product31/3
  [xi_pesai_x_b1_2] -> Product127/2
  [k_c_l2_2] -> Product58/1  "k_c_l2"
  [shangjie_yuzhi_2] -> Add68/3
  Add70/1 -> [u_l_1_2], Scope62/1
  [k_ke_xi_l_2] -> Product109/2  "k_ke_xi_l"
  Product120/1 -> Integrator4/1
  [c2_l_2] -> Add133/3
  Product31/1 -> Gain33/1
  [z_pesai_2] -> Product61/1
  [yipuxilong_pesai_2] -> Add61/2
  Subtract3/1 -> Divide41/1
  [theta_id_2] -> Add18/3
  Product80/1 -> Add133/2
  Add13/1 -> Product63/1
  [pesai_jie_a1_2] -> Scope229/2, MATLAB Function4/3(jie)
  Product125/1 -> Scope1/1, Add140/1
  Product57/1 -> Add65/2
  Add16/1 -> Scope223/2, [oumiga_id_2], Integrator29/1
  [xi_l_2] -> Product60/3
  Gain8/1 -> [u_21_2]
  Product61/1 -> Add64/4
  MATLAB Function7/2(a) -> Scope212/1, Multiport Switch1/1
  Integrator4/1 -> To Workspace3/1, Scope382/1, [x2]  "xi"
  [yita_l_2] -> Math Function14/1
  [ke_xi_pesai_2] -> Derivative38/1
  [c2_pesai_2] -> Add71/3
  [yipuxilong_l_2] -> Derivative7/1
  [pesai_2] -> Subtract6/1
  Derivative45/1 -> Saturation14/1
  Switch8/1 -> Switch12/3
  Math Function10/1 -> Product58/2
  Switch11/1 -> Scope210/1, Scope216/1, Memory17/1, Scope211/1
  [shangjie_yuzhi_2] -> MATLAB Function7/6(shangjie_yuzhi)
  Constant153/1 -> Gain16/1
  Memory4/1 -> MATLAB Function15/7(d1_dotb)
  [l_ni2_2] -> Divide17/2
  [oumiga_L] -> Add129/1
  Integrator21/1 -> Scope182/1
  [pesai_d1_2] -> Switch11/3
  [oumiga_L_dot] -> Divide11/3
  Trigonometric Function8/1 -> Product19/2
  [yita_l_2] -> Math Function34/1
  [c2_pesai_2] -> Add65/3
  Add18/1 -> Trigonometric Function9/1
  [ke_xi_l_2] -> Derivative6/1
  [e_pesai_2] -> Product57/2
  Trigonometric Function7/1 -> Product21/2
  [xiajie_yuzhi_2] -> MATLAB Function17/2(xiajie_yuzhi)
  Trigonometric Function10/1 -> Divide12/3
  [c3_l_2] -> Product112/1
  Gain18/1 -> Add54/3
  Divide8/1 -> Subtract3/6
  [fai_2] -> Trigonometric Function16/1
  [k_ke_xi_l_dot_2] -> Product26/2
  Divide6/1 -> Subtract3/5
  [theta_L] -> Subtract6/3
  [fai_2] -> Subtract20/1
  [pesai_d1_2] -> Switch12/1
  Add57/1 -> Product65/2
  Product65/1 -> Math Function6/1
  [ke_xi_l_dot_2] -> Product81/3
  [xi_pesai_0_2] -> MATLAB Function4/1(x0)
  [e_l_dot_2] -> Add133/1
  Add36/1 -> Integrator17/1
  [l_ni1_2] -> Divide41/2
  [vL] -> Divide42/1
  [oumiga_L] -> Product20/1
  Add4/1 -> Scope178/1, [xi_pesai_0_xia_2]
  MATLAB Function4/2(a) -> Scope232/1
  [yita_l_2] -> Add53/1
  Derivative7/1 -> [yipuxilong_l_dot_2]
  [xi_pesai_dot_2] -> Product64/1
  [h] -> MATLAB Function10/4(h)
  [row_wuqiong_2] -> Add13/2
  [xi_l_2] -> Derivative41/1
  [rou_0_2] -> Gain44/1, Product128/2, Add142/1
  Product82/1 -> Add60/3
  Product70/1 -> [ke_xi_l_2]
  [fai_d_2] -> Subtract20/2
  [e_l_2] -> Product68/1
  MATLAB Function16/2(a) -> Scope55/1
  MATLAB Function17/3(d1_fn) -> [pesai_fin_b1_2]
  [c1_pesai_2] -> Divide2/1
  Math Function13/1 -> Scope171/1, Add47/2
  Math Function11/1 -> Product28/2
  [h] -> Divide11/1
  Add40/1 -> Scope168/1, Product49/3
  Add48/1 -> Scope213/1, [xi_pesai_0_2]
  [u_11_2] -> Add29/1
  Add54/1 -> Product117/1, [xi_pesai_2], Scope96/1
  [k_ke_xi_l_2] -> Product81/2  "k_ke_xi_l"
  [x2] -> Add19/2
  Constant95/1 -> Gain18/1
  Integrator3/1 -> To Workspace8/1, Scope383/1, [y2]  "yi"
  [pesai_2] -> Trigonometric Function22/1
  Divide13/1 -> Subtract17/6
  [fai_2] -> Trigonometric Function31/1
  Square1/1 -> [l_ni2_2], Scope97/1
  [c1_pesai_2] -> Product27/2, Scope134/1
  [theta_2] -> Add21/1
  [theta_2] -> Scope81/2
  Product21/1 -> Add16/1
  Math Function12/1 -> Add46/2
  Gain16/1 -> Add68/2
  [k_yita_pesai_2] -> Product78/1  "k_yita_pesai"
  [xi_pesai_0_xia_2] -> MATLAB Function17/1(x0)
  [e_l_2] -> Product112/2
  [theta_L] -> Add68/1
  [z_l_2] -> Product26/1
  [theta_L] -> Add17/1
  [theta_2] -> Subsystem2/6(In6)
  Sin5/1 -> Product122/2
  Trigonometric Function26/1 -> Divide7/3
  Derivative29/1 -> Saturation15/1
  Constant72/1 -> Math Function9/2
  [theta_id_2] -> Add126/3
  Subtract19/1 -> Scope93/1, [gama_2]
  Product18/1 -> Add19/1
  [pesai_d1_00_a1_2] -> Scope233/1, Add135/3
  [yita_pesai_2] -> Add61/1
  [oumiga_2] -> Add127/3, Scope151/1
  Product75/1 -> [c2_l_2]
  Integrator30/1 -> Scope384/1, [theta_2]  "theta_i"
  Integrator17/1 -> Math Function11/1, Scope173/1, [c_d_pesai_2]
  [xiajie_yuzhi_2] -> Add139/2
  [y2] -> Add25/2
  [xi_pesai_0_2] -> MATLAB Function15/1(x0)
  Gain31/1 -> Product39/2
  Trigonometric Function1/1 -> MATLAB Function10/1(s)
  Add41/1 -> Product49/4
  [pesai_2] -> Trigonometric Function32/1
  Memory12/1 -> Switch8/1
  Subtract10/1 -> Scope129/1, [e_l_2]
  [xF2head] -> Subsystem2/8(In8)
  Product124/1 -> Add142/2
  [fai_d_2] -> Add20/3
  Gain44/1 -> Add141/2
  Product122/1 -> Scope56/1, Add135/1
  Constant99/1 -> Subtract6/4
  Math Function7/1 -> Product81/1
  MATLAB Function15/2(d1_dot) -> [pesai_d1_dot_a1_2]
  Product27/1 -> Gain32/1
  Trigonometric Function20/1 -> Divide16/2
  [l_dot_2] -> Divide17/3
  MATLAB Function17/1(d1) -> [pesai_d1_00_b1_2]
  Product49/1 -> Scope181/1, [ke_xi_pesai_2]
  [l_2] -> MATLAB Function10/3(l)
  [k_row_2] -> Product52/1
  [ke_xi_l_dot_3] -> ?
  [xiajie_yuzhi_3] -> ?
  ? -> ?
  [shang_] -> ?
  Trigonometric Function74/1 -> Divide58/2
  Divide43/1 -> Saturation11/1
  [e_pesai_dot_3] -> Add188/1
  Constant130/1 -> Gain38/1
  [pesai_d_b1_3] -> Scope348/1, Multiport Switch2/3
  [ke_xi_l_3] -> Derivative12/1
  Product131/1 -> Scope247/1, Add179/4
  Constant79/1 -> Math Function35/2
  Subtract23/1 -> Divide62/1
  [yipuxilong_pesai_dot_3] -> Product151/1
  [fai_3] -> Trigonometric Function62/1
  [fai_3] -> MATLAB Function22/3(fai)
  [d] -> Product48/4
  Integrator42/1 -> Scope297/1
  Saturation11/1 -> Product140/1
  Add190/1 -> Scope371/1, Product152/2
  Product155/1 -> Add194/1
  MATLAB Function14/2(W) -> Scope236/1, [oumiga_3_dot_liju], Integrator35/1
  Add27/1 -> [z_l_3]
  [xia] -> Add239/4
  Gain79/1 -> Add239/3
  Divide61/1 -> Subtract22/4
  [xi_pesai_x_b1_3] -> Product197/2
  Product191/1 -> Add226/2
  [h] -> Divide53/1
  Gain54/1 -> Scope200/1, [u_22_3]
  [oumiga_3] -> Divide60/3
  [xi_pesai_3] -> Product185/1
  [oumiga_3] -> MATLAB Function22/5(oumiga_i)
  Trigonometric Function65/1 -> Divide63/2
  [xiajie_yuzhi_3] -> MATLAB Function37/5(xiajie_yuzhi)
  Gain51/1 -> Product140/2
  [c3_pesai_3] -> Product179/2
  [xi_l_3] -> Product161/3
  [theta_3] -> Subtract25/2
  [fai_d_3] -> Add235/1
  [pesai_fin_b1_3] -> Scope388/3, MATLAB Function37/4(fin)
  [theta_1] -> Add191/1
  [pesai_d_a1_3] -> Multiport Switch2/2
  [xF3head] -> Subsystem5/8(In8)
  [fai_3] -> Trigonometric Function74/1
  Product157/1 -> Math Function38/1
  Divide55/1 -> Subtract23/1
  Add153/1 -> [xi_pesai_0_shang_3_qiehuan]
  [xi_pesai_x_b1_3] -> Product194/2
  Product140/1 -> Scope196/1, Add157/3
  Derivative8/1 -> MATLAB Function38/4(d1_dotu)
  Subsystem5/2(Out3) -> [xia], Scope423/1, [pesai_4]
  [oumiga_1] -> Divide48/2
  [c1_l_3] -> Divide54/1
  [h] -> MATLAB Function22/7(h)
  Add26/1 -> Add153/2
  [pesai_d1_3] -> Add153/1
  [c1_l_3] -> Product163/2
  Constant141/1 -> Gain50/1
  Constant137/1 -> Add26/5
  [pesai_d1_00_a1_3] -> Scope411/1, Add224/3
  [k_c_pesai2_3] -> Product133/1
  [yF1head] -> Subsystem3/4(In4)
  [c3_l_3] -> Product173/1
  MATLAB Function38/1(d1) -> Scope413/1, [pesai_d1_00_b1_3]
  [yipuxilong_pesai_3] -> Add158/1
  Add225/1 -> [k_tiaota_a1_3]
  [h] -> Divide47/1
  [pesai_dot_3] -> Scope421/2
  Derivative43/1 -> [c1_l_dot_3]
  [theta_3] -> Add191/3
  Divide45/1 -> Subtract23/3
  [xia] -> Add235/4
  [xi_pesai_3] -> Scope261/1, Product143/2
  [x3] -> Add145/2
  Math Function37/1 -> Add158/2
  [yF3head] -> Subsystem5/5(In5)
  Divide44/1 -> Scope240/1, Square3/1, [l_ni1_3]  "求逆"
  [xF2head] -> Subsystem5/7(In7)
  Subsystem5/1(seita_i) -> Scope424/1
  [yF2head] -> Subsystem5/4(In4)
  MATLAB Function37/2(a) -> Scope391/1
  Derivative64/1 -> MATLAB Function36/4(d1_dotu)
  [xF2head] -> Subsystem5/2(In2)
  [yF3head] -> Subsystem5/10(In10)
  [d] -> Product74/1
  [pesai_3] -> Trigonometric Function52/1
  [fai_d_3] -> Add151/1
  Constant298/1 -> Gain79/1
  MATLAB Function38/2(d1_dot) -> Scope414/1, [pesai_d1_dot_b1_3]
  [v3] -> Product181/2, Product180/1
  [fai_d_3] -> Add239/1
  Product150/1 -> Add186/2
  Product194/1 -> Add232/2
  [pesai_jie_b1_3] -> Scope388/2, MATLAB Function37/3(jie)
  Constant297/1 -> Add237/5
  Add237/1 -> Add238/1
  Product62/1 -> Add51/1
  [pesai_d1_3] -> Add200/2
  Constant268/1 -> Add200/3
  [pesai_d1_3] -> Add236/1
  [fai_dot_3] -> Subtract21/1
  Add238/1 -> [pesai_d_b1_3]
  Gain38/1 -> Add26/3
  [xF3head] -> Foolower_3/3(xf1head)
  Add144/1 -> Trigonometric Function59/1
  Constant295/1 -> Add235/5
  [yita_l_3] -> Math Function46/1
  [rou_0_3] -> Add232/1
  [shangjie_yuzhi_3] -> Add223/1
  [oumiga_1] -> Divide61/3
  [theta_id_3] -> Add171/1
  Constant294/1 -> Gain77/1
  [xiajie_yuzhi_3] -> MATLAB Function38/2(xiajie_yuzhi)
  [theta_1] -> Add171/2
  Product137/1 -> Gain53/1
  Gain77/1 -> Add235/3
  [k_tiaota_a1_3] -> Product193/1
  [xF3head] -> Subsystem5/3(In3)
  Constant273/1 -> Gain46/1
  [theta_1] -> Add192/1
  Derivative61/1 -> Saturation23/1
  [pesai_d_a1_3000] -> Add152/2
  [xi_pesai_x_b1_3] -> Add233/2
  Foolower_3/1(ldot) -> [l_3], Scope244/1
  Add193/1 -> Add168/1, Scope265/1, Integrator42/1
  Gain75/1 -> Sin10/1
  Gain71/1 -> Sin9/1
  [xi_pesai_0_shang_3_qiehuan] -> MATLAB Function36/1(x0)
  MATLAB Function36/1(d1) -> [pesai_d1_00_a1_3]
  Product197/1 -> Scope389/1, Add230/2
  Product198/1 -> Scope390/1, [xi_pesai_x_b1_3]
  Constant275/1 -> Gain56/1
  Gain76/1 -> Add231/2
  Product180/1 -> Integrator32/1
  [y3] -> Add150/2
  [oumiga_3] -> MATLAB Function23/5(oumiga_i)
  [xia] -> Add237/4
  [k_tiaota_b1_3] -> Product197/1
  [xi_pesai_x_a1_3] -> Add227/2
  [xia_] -> ?
  MATLAB Function36/2(d1_dot) -> Scope285/1, [pesai_d1_dot_a1_3]
  [xi_pesai_0_shang_3_qiehuan] -> Scope405/1, MATLAB Function39/2(d1), MATLAB Function39/1(x0)
  Constant293/1 -> Add233/1
  [theta_1] -> Subtract25/3
  [oumiga_3] -> Divide52/2
  [c1_pesai_3] -> Product141/1
  [theta_3] -> Scope202/2
  Clock6/1 -> Gain57/1
  Math Function46/1 -> Add190/2
  [pesai_d1_dot_b1_3] -> Memory41/1
  Constant271/1 -> Gain65/1
  Gain52/1 -> Scope199/1, [u_12_3]
  Add224/1 -> [pesai_jie_a1_3], Scope404/1
  [pesai_d1_dot_a1_3] -> Add225/1
  [k_ke_xi_pesai_dot_3] -> Product153/2
  [u_l_1_3] -> MATLAB Function14/5(u1)
  Memory38/1 -> MATLAB Function36/7(d1_dotb)
  Derivative62/1 -> Add240/2, Scope420/1
  Divide54/1 -> Saturation16/1
  Subtract21/1 -> Scope241/1
  [pesai_d1_00_a1_3] -> Memory37/1
  [xi_pesai_0_shang_3_qiehuan] -> Derivative64/1, MATLAB Function36/3(d1u), MATLAB Function36/5(d1_fnu)
  MATLAB Function39/1(y) -> Add228/1, Derivative61/1, Scope403/1
  [c1_pesai_3] -> Divide43/1
  [c1_l_3] -> Derivative43/1
  [rou_0_3] -> Product196/2
  Derivative20/1 -> [c1_pesai_dot_3]
  Product196/1 -> Scope409/1, [xi_pesai_x_a1_3]
  [shangjie_yuzhi_3] -> MATLAB Function39/5(shangjie_yuzhi)
  Constant299/1 -> Add239/5
  Add227/1 -> Gain71/1
  Product135/1 -> Gain67/1
  [fai_d_3] -> Add237/1
  [h] -> Divide60/1
  Product133/1 -> Add160/2, Scope192/1
  [oumiga_3] -> Scope324/1
  Saturation23/1 -> Scope412/1
  [fai_3] -> Trigonometric Function71/1
  Memory37/1 -> MATLAB Function36/6(d1b)
  Memory41/1 -> MATLAB Function38/7(d1_dotb)
  [yF2head] -> Subsystem5/9(In9)
  Math Function45/1 -> Scope269/1, Add170/2
  Cos12/1 -> Product74/2
  Add177/1 -> Product161/4
  MATLAB Function36/3(d1_fn) -> [pesai_fin_a1_3]
  [pesai_d1_dot_b1_3] -> Add231/1
  Add228/1 -> [pesai_d_a1_3000]
  [pesai_d_3] -> Add204/2
  Add231/1 -> [k_tiaota_b1_3]
  Constant80/1 -> Subtract25/4
  Product170/1 -> Scope191/1, Add27/2
  MATLAB Function39/2(a) -> Scope410/1
  Sin9/1 -> Product192/2
  Saturation16/1 -> Product168/1
  [row_0_3] -> Add38/1
  [xi_l_3] -> Product152/3
  Subtract29/1 -> Scope208/1, [gama_3]
  Product74/1 -> Add150/1
  MATLAB Function8/2(a) -> Scope281/1, [a], Multiport Switch2/1
  Constant276/1 -> Add205/5
  [xi_xia] -> Scope311/2
  Add236/1 -> [xi_pesai_0_xia_3_qiehuan]
  Add166/1 -> Product157/1
  Add170/1 -> Scope239/1, Product151/4
  [pesai_d_3] -> Add205/2
  [pesai_d000] -> Scope128/3
  Add204/1 -> Scope339/1, Scope283/1, [xi_pesai_3]
  [xi_shang] -> Scope283/2
  [shang] -> Add26/4
  [fai_3] -> Trigonometric Function68/1
  [h] -> Divide52/1
  [fai_d_3] -> Add205/1
  [shang] -> Add204/4
  Constant274/1 -> Add204/5
  [xF1head] -> Subsystem3/2(In2)
  Gain46/1 -> Add204/3
  [yipuxilong_pesai_3] -> Scope268/1, Add170/1
  [pesai_d1_3] -> Scope314/1, MATLAB Function8/1(d1)
  [xiajie_yuzhi_3] -> Add201/2
  MATLAB Function23/1(y) -> Scope300/1
  Constant200/1 -> Add191/4
  [xia] -> Add201/4
  [yipuxilong_l_3] -> Add178/2
  [yita_pesai_3] -> Math Function44/1
  [fai_d_3] -> Gain64/1
  Constant270/1 -> Gain45/1
  [v3] -> MATLAB Function23/2(Vi)
  [z_pesai_3] -> Product141/2
  Gain39/1 -> Add185/3
  [shang] -> Add185/4
  Add191/1 -> Scope266/2, Add196/1, Scope322/1
  Trigonometric Function61/1 -> Divide51/2
  Divide51/1 -> Subtract28/5
  Math Function43/1 -> Product133/2
  [theta_id_3] -> Add144/3
  [pesai_fin_a1_3] -> Memory40/1
  Add179/1 -> Product163/1
  Add174/1 -> Product159/4
  Derivative52/1 -> [xi_pesai_dot_3]
  [oumiga_3] -> Integrator45/1
  Add51/1 -> Scope324/2, [oumiga_id_3], Integrator44/1
  Add151/1 -> Add152/1
  MATLAB Function38/4(a) -> Scope417/1
  Subtract25/1 -> [fai_3], Scope315/1
  [e_pesai_3] -> Scope262/1, Product143/1
  Divide62/1 -> Subtract24/2
  Integrator35/1 -> [oumiga_3], Scope194/1
  [oumiga_3] -> Add197/2
  Add184/1 -> Product147/1
  [pesai_dot_3] -> Divide47/4
  [fai_3] -> Trigonometric Function64/1
  Add200/1 -> [beta_3], Scope270/2
  Trigonometric Function69/1 -> Divide48/3
  Constant160/1 -> Add173/1
  Integrator44/1 -> [theta_id_3], Scope202/1, Scope295/1
  Add44/1 -> Trigonometric Function58/1
  Math Function48/1 -> Scope242/1, Product164/4
  Divide49/1 -> Subtract28/2
  [yita_pesai_3] -> Add164/1
  [e_l_dot_3] -> Add198/1
  [theta_id_3] -> Add44/2
  [oumiga_1] -> MATLAB Function22/6(oumiga_L)
  Divide48/1 -> Subtract23/6
  [z_l_3] -> Product169/1
  Product165/1 -> Add179/1
  [xi_pesai_3_xia] -> Product185/2
  [theta_id_3] -> Add192/3
  Math Function42/1 -> Product150/2
  [fai_3] -> Trigonometric Function69/1
  [fai_3] -> Trigonometric Function72/1
  [xi_pesai_x_a1_3] -> Product191/2
  [fai_d_3] -> Add144/1
  [theta_id_3] -> Add28/1
  MATLAB Function38/3(d1_fn) -> Scope415/1, [pesai_fin_b1_3]
  From1047/1 -> Product135/2
  [yipuxilong_l_dot_3] -> Product161/1
  [ke_xi_pesai_3] -> Math Function50/1
  Trigonometric Function55/1 -> Product180/2
  [shang] -> Add151/4
  [z_pesai_3] -> Divide43/2
  [yita_l_3] -> Add176/1
  Constant175/1 -> Math Function40/2
  Trigonometric Function51/1 -> MATLAB Function14/1(s)
  [theta_3] -> Subsystem3/6(In6)
  [oumiga_1] -> Scope248/1, Add193/1
  [row_wuqiong_3] -> Add194/2
  [pesai_d_b1_3000] -> Add238/2
  [rou_0_3] -> Gain76/1
  Add171/1 -> Scope270/1
  Add230/1 -> [pesai_jie_b1_3], Scope387/1
  Product195/1 -> Scope378/1, Add230/1
  Add198/1 -> Product172/1
  [c1_pesai_3] -> Product147/2
  [pesai_d1_3] -> Scope348/2, Multiport Switch2/4
  [e_l_dot_3] -> Add199/1
  Subsystem3/1(seita_i) -> Scope328/1
  [c1_pesai_3] -> Product132/2, Scope255/1
  Gain57/1 -> Product148/2
  [oumiga_1] -> Add195/1
  Add59/1 -> Trigonometric Function57/1
  Integrator43/1 -> [v3], Scope190/1
  [oumiga_3] -> Add193/3, Scope264/1
  [oumiga_3] -> Subtract26/2
  [fai_d_3] -> Add185/1
  Product48/1 -> Add51/3
  [yF3head] -> Subsystem3/10(In10)
  Math Function35/1 -> Scope325/1, Product139/2
  [rou_0_3] -> Product198/2
  Gain53/1 -> Scope253/1, Add183/2
  [vL_dot_1] -> Divide56/1
  Subtract22/1 -> Divide57/1
  Derivative14/1 -> [yipuxilong_l_dot_3]
  [k_tiaota_b1_3] -> Product194/1
  Add181/1 -> Scope293/1, Gain30/1
  [c2_l_3] -> Add199/3
  Constant192/1 -> Divide44/1
  Constant162/1 -> Math Function43/2
  [theta_3] -> Trigonometric Function54/1
  Add154/1 -> [u_pesai_1_3], Scope310/1
  Trigonometric Function62/1 -> Divide53/3
  [pesai_3] -> Trigonometric Function53/1
  [l_3] -> MATLAB Function22/8(L)
  [l_ni1_3] -> Divide62/2
  [k_row_3] -> Product148/1
  [yipuxilong_l_3] -> Add177/1
  Constant144/1 -> Add151/5
  [fai_d_3] -> Add26/1
  [oumiga_id_3] -> Add197/3
  Subtract24/1 -> Add157/1
  [fai_3] -> Derivative50/1
  Math Function40/1 -> Product170/1
  Trigonometric Function54/1 -> Product181/1
  [xi_pesai_3] -> Product156/2
  [c2_pesai_3] -> Add184/3
  Gain72/1 -> Add225/2
  Add205/1 -> Scope347/1, Scope311/1, [xi_pesai_3_xia]
  [fai_3] -> Trigonometric Function61/1
  Integrator33/1 -> To Workspace11/1, [x3], Scope419/1  "xi"
  [c3_l_3] -> Product162/2
  [e_pesai_3] -> Product136/2
  [fai_3] -> Add191/2
  Add194/1 -> Gain69/1, Scope193/1, [xi_l_3]
  Constant169/1 -> [row_wuqiong_3]
  [l_3] -> Subtract27/1
  [h] -> MATLAB Function14/4(h)
  Multiport Switch2/1 -> Scope349/1, [pesai_d000], [pesai_d_3]
  Product179/1 -> Add157/2, Scope201/1
  [e_l_3] -> Product166/2
  [xF1head] -> Foolower_3/1(xl)
  [yita_l_3] -> Add178/1
  [yipuxilong_l_3] -> Add190/1
  [theta_1] -> Add148/2
  Product25/1 -> Add145/1
  Cos11/1 -> Product25/2
  Derivative12/1 -> [ke_xi_l_dot_3], Scope204/1
  Add175/1 -> Product178/1, Goto243/1, Scope237/1
  Add192/1 -> [pesai_d1_3], Scope323/1
  [vL_dot_1] -> Divide55/1
  Gain49/1 -> [u_11_3], Scope275/1
  [e_l_dot_3] -> Product162/1
  [xia] -> Add205/4
  [oumiga_3] -> Subtract21/3
  MATLAB Function36/4(a) -> Scope282/1
  Add234/1 -> [pesai_d_b1_3000]
  [rou_0_3] -> Gain72/1
  [pesai_d1_00_b1_3] -> Scope401/1, Add230/3
  [xi_pesai_x_a1_3] -> Product193/2
  [k_tiaota_a1_3] -> Product191/1
  [yF1head] -> Foolower_3/2(yl)
  Constant267/1 -> Gain39/1
  MATLAB Function22/1(y) -> Scope299/1
  [xi_l_3] -> Product158/2
  [pesai_d_3] -> Add196/2, Scope278/1
  [yita_l_3] -> Add174/1
  Add239/1 -> Derivative62/1
  Product163/1 -> Gain54/1
  [theta_1] -> Add146/1
  [h] -> Divide61/1
  Add173/1 -> Product159/3
  Product173/1 -> Add198/2
  [yipuxilong_l_3] -> Derivative14/1
  [e_pesai_dot_3] -> Product179/1
  Derivative57/1 -> [e_l_dot_3]
  Math Function47/1 -> Add176/2
  Constant172/1 -> Add166/1
  [theta_id_3] -> Add149/1
  [k_ke_xi_pesai_3] -> Product144/2  "k_ke_xi_pesai"
  [theta_3] -> Cos12/1
  [fai_3] -> Trigonometric Function63/1
  Add160/1 -> Integrator39/1
  Constant171/1 -> [yipuxilong_l_3]
  [oumiga_1] -> Divide53/2
  [u_11_3] -> Add154/1
  Add189/1 -> Scope292/1, [z_pesai_3]
  [pesai_3] -> Subtract25/1
  Product151/1 -> [c2_pesai_3]
  Trigonometric Function73/1 -> Divide50/2
  Add226/1 -> Product192/1
  Gain78/1 -> Add237/3
  Trigonometric Function71/1 -> Divide55/2
  Trigonometric Function52/1 -> Divide59/2
  [yita_l_3] -> Add173/2
  [l_d_3] -> Subtract27/2
  Integrator34/1 -> Subtract29/2
  [fai_dot_3] -> Divide49/3
  [yF3head] -> Subsystem3/5(In5)
  Integrator39/1 -> Math Function43/1, Scope271/1, [c_d_pesai_3]
  [z_pesai_3] -> Product153/1
  Integrator45/1 -> [theta_3]  "theta_i"
  [yita_l_3] -> Add166/2
  [yita_pesai_3] -> Add163/2
  [oumiga_1] -> MATLAB Function23/6(oumiga_L)
  Constant147/1 -> Math Function50/2
  [yita_pesai_3] -> Product146/2
  Divide50/1 -> Subtract28/3
  Gain61/1 -> Goto290/1, Scope246/1
  Divide53/1 -> Subtract28/6
  [u_12_3] -> Add154/2
  Subtract26/1 -> Integrator34/1
  [fai_3] -> Subtract29/1
  [u_pesai_1_3] -> MATLAB Function14/6(u2)
  [c1_pesai_3] -> Derivative20/1
  Add233/1 -> Gain75/1
  [e_l_3] -> Derivative57/1
  Trigonometric Function72/1 -> Divide49/2
  Add164/1 -> Product146/4
  [fai_d_3] -> Add200/1
  [fai_d_3] -> Add192/2
  [yF1head] -> Subsystem3/9(In9)
  [oumiga_L_dot_1] -> Divide46/3
  Trigonometric Function68/1 -> Divide46/2
  Add187/1 -> [u_l_1_3], Scope187/1
  Subsystem3/2(Out3) -> Scope256/1, Derivative66/1, [shang], [pesai_3]
  [k_yita_pesai_3] -> Product164/1  "k_yita_pesai"
  [theta_1] -> Add28/2
  Derivative56/1 -> [xi_l_dot_3]
  [z_l_3] -> Math Function35/1
  MATLAB Function37/1(y) -> Add234/1, Derivative63/1, Scope379/1
  Product142/1 -> [c3_l_3]
  [theta_id_3] -> Add59/2
  [xi_pesai_0_xia_3_qiehuan] -> Scope345/1, Derivative8/1
  Product167/1 -> Gain55/1
  [v1] -> Divide58/1
  [v1] -> MATLAB Function23/1(VL)
  [xia] -> ?
  [z_l_3] -> Product131/1
  [xi_pesai_3] -> Product151/3
  [theta_1] -> Add175/2
  [e_l_3] -> Product173/2
  [fai_d_3] -> Add204/1
  Constant155/1 -> Gain48/1
  [ke_xi_l_dot_3] -> Product167/3
  Add148/1 -> Product178/2, Scope243/1
  [yita_l_3] -> Math Function51/1
  Constant189/1 -> Add146/4
  Divide60/1 -> Subtract22/3
  Add195/1 -> [pesai_d1_3_dot], Add168/2, Integrator41/1
  [xF3head] -> Subsystem3/8(In8)
  [yipuxilong_pesai_3] -> Add164/2
  [yita_pesai_3] -> Math Function45/1
  Constant110/1 -> Goto263/1
  [c2_l_3] -> Add198/3
  Gain55/1 -> Add179/2
  [theta_id_3] -> Add146/2
  Add145/1 -> [xF3head]
  Derivative63/1 -> Saturation26/1
  Product193/1 -> Scope408/1, Add224/2
  Product164/1 -> Scope259/1, [c1_pesai_3]
  [oumiga_3] -> Divide47/2
  [u_21_3] -> Add187/1
  Subtract27/1 -> Scope251/1, [e_l_3]
  [k_ke_xi_l_3] -> Product170/2  "k_ke_xi_l"
  Add149/1 -> Scope206/1
  [shangjie_yuzhi_3] -> Add185/2
  [yipuxilong_pesai_3] -> Add182/2
  [pesai_d1_00_b1_3] -> Memory39/1
  Product159/1 -> [ke_xi_l_3]
  [fai_d_3] -> Add146/3
  MATLAB Function14/1(V) -> [v3_dot_liju], Integrator43/1, Scope235/1
  Product166/1 -> Add199/2
  [theta_3] -> Subsystem3/1(In1)
  Trigonometric Function58/1 -> Product32/2
  Add188/1 -> Product134/1
  Derivative54/1 -> Scope306/1, [ke_xi_pesai_dot_3]
  Product162/1 -> Add181/2
  [ke_xi_l_3] -> Math Function39/1
  Constant177/1 -> Add162/1
  Sin10/1 -> Product195/2
  Add38/1 -> Product155/1
  Add186/1 -> Integrator40/1
  Gain56/1 -> Add205/3
  Product149/1 -> Add184/2
  Product143/1 -> Scope260/1, [yita_pesai_3]
  [fai_dot_3] -> Add193/2, Scope263/1
  Product139/1 -> Add179/3
  [k_yita_l_3] -> Scope370/1, Product152/1  "k_yita_l"
  [c3_pesai_3] -> Product136/1
  Add28/1 -> Scope245/1
  [xi_pesai_3] -> Derivative52/1
  Math Function36/1 -> Product155/2
  [xi_l_3] -> Derivative56/1
  [yipuxilong_pesai_3] -> Derivative55/1
  Constant201/1 -> Add192/4
  [d] -> Product25/1
  Divide46/1 -> Subtract23/5
  [pesai_3] -> Scope266/1
  Gain67/1 -> Scope336/1
  [xi_pesai_0_xia_3_qiehuan] -> Scope416/1, Add229/1
  Divide58/1 -> Subtract22/1
  Product136/1 -> Add188/2
  [l_3] -> Divide44/2
  Trigonometric Function60/1 -> Divide52/3
  Divide63/1 -> Subtract23/2
  Constant103/1 -> Goto325/1
  [c1_l_3] -> Product169/3
  Divide59/1 -> Subtract22/2
  [theta_1] -> Add59/1
  [yita_pesai_3] -> Add162/2
  [fai_dot_3] -> Divide63/3
  Add168/1 -> Scope326/1
  [c1_l_3] -> Product172/2
  Add197/1 -> Scope290/1
  Constant269/1 -> Add185/5
  Trigonometric Function57/1 -> Product62/2
  Product134/1 -> Scope252/1, Add183/1
  [u_22_3] -> Add187/2
  MATLAB Function8/1(d) -> Scope128/1, Scope316/1
  Math Function51/1 -> Add177/2
  [xF3head] -> Subsystem3/3(In3)
  [c_d_l_3] -> Product168/2  "自适应参数"
  [theta_1] -> Add44/1
  [oumiga_id_3] -> Add195/2
  [xi_pesai_0_xia_3_qiehuan] -> MATLAB Function38/3(d1u), MATLAB Function38/5(d1_fnu)
  Saturation26/1 -> Scope402/1
  [xi_pesai_3] -> Product164/3
  Product147/1 -> Scope294/1, Add189/1
  [h] -> Divide51/1
  Add152/1 -> [pesai_d_a1_3]
  Trigonometric Function53/1 -> Divide60/2
  [pesai_fin_a1_3] -> Scope405/3, MATLAB Function39/4(fin)
  [pesai_d1_dot_a1_3] -> Memory38/1
  Add235/1 -> Add236/2
  [e_l_3] -> Product158/1
  [ke_xi_pesai_dot_3] -> Product137/3
  [h] -> Divide46/1
  [fai_3] -> Subtract30/1
  Memory40/1 -> MATLAB Function36/8(d1_fnb)
  Trigonometric Function66/1 -> Divide45/2
  [theta_id_0_3] -> Add175/1
  Subtract30/1 -> Scope320/1, Derivative47/1
  [xi_pesai_0_xia_3_qiehuan] -> MATLAB Function38/1(x0)
  [l_d_3] -> Product48/3
  [xi_pesai_dot_3] -> Product156/1
  [theta_3] -> Subsystem5/6(In6)
  [v1] -> MATLAB Function22/1(VL)
  [theta_3] -> Subsystem5/1(In1)
  Product148/1 -> Math Function36/1
  Product178/1 -> Gain61/1
  [pesai_3] -> Trigonometric Function66/1
  [yita_pesai_3] -> Math Function37/1
  Divide56/1 -> Subtract28/1
  [k_z_l_3] -> Product139/1
  Derivative50/1 -> [fai_dot_3], Scope321/2
  [xF1head] -> Subsystem3/7(In7)
  [yipuxilong_l_3] -> Add174/2
  [pesai_3] -> MATLAB Function22/4(pesai)
  Add147/1 -> Scope189/1
  Constant296/1 -> Gain78/1
  [pesai_dot_3] -> Divide45/3
  [fai_d_3] -> Subtract30/2
  Product146/1 -> Scope279/1, [ke_xi_pesai_3]
  Product144/1 -> Scope301/1, Add189/2
  [oumiga_1] -> Subtract21/2
  Math Function50/1 -> Product144/1
  [l_3] -> MATLAB Function14/3(l)
  [pesai_dot_3] -> Divide52/4
  [k_c_l_3] -> Product169/2  "k_c_l"
  [pesai_d1_3] -> Scope128/2
  Product32/1 -> Add51/2
  Gain45/1 -> Add201/3
  Trigonometric Function67/1 -> Divide47/3
  Product156/1 -> [c3_pesai_3]
  [fai_dot_3] -> Divide53/4
  [k_ke_xi_l_3] -> Product167/2  "k_ke_xi_l"
  Product158/1 -> Scope369/1, [yita_l_3]
  [ke_xi_pesai_3] -> Derivative54/1
  Product161/1 -> [c2_l_3]
  Math Function44/1 -> Add169/2
  [xi_pesai_0_xia_3_qiehuan] -> Scope388/1, MATLAB Function37/2(d1)
  [k_ke_xi_l_dot_3] -> Product131/2
  Math Function38/1 -> Product152/4
  [theta_3] -> Add149/2
  [k_c_pesai_3] -> Product141/3  "k_c_pesai"
  Gain48/1 -> Add148/3
  [theta_1] -> Add144/2
  Memory36/1 -> MATLAB Function38/8(d1_fnb)
  [theta_3] -> Add147/1
  Subtract28/1 -> Add181/1
  Add169/1 -> Product151/2
  [e_pesai_3] -> Derivative53/1
  [oumiga_1] -> Product62/1
  Integrator32/1 -> To Workspace12/1, [y3], Scope428/1  "yi"
  [k_ke_xi_pesai_3] -> Product137/2  "k_ke_xi_pesai"
  [pesai_3] -> MATLAB Function23/4(pesai)
  [theta_id_0_3] -> Add148/1
  Trigonometric Function56/1 -> MATLAB Function14/2(c)
  Product152/1 -> Scope368/1, [c1_l_3]
  [theta_3] -> Subsystem3/11(In11)
  [v3] -> Divide45/1
  [theta_id_3] -> Add147/2
  Constant170/1 -> [row_0_3]
  [pesai_dot_3] -> Divide50/3
  [theta_3] -> Cos11/1
  [row_wuqiong_3] -> Add38/2
  Integrator40/1 -> Math Function42/1, Scope319/1, [c_d_l_3]
  [d] -> Product32/3
  Add162/1 -> Scope273/1, Product24/1
  Constant145/1 -> Add163/1
  [l_dot_3] -> Divide57/3
  Math Function49/1 -> Product137/1
  [e_pesai_dot_3] -> Add184/1
  Product23/1 -> Add183/3
  [pesai_3] -> Trigonometric Function56/1, Trigonometric Function51/1
  [v1] -> Divide49/1
  [c2_pesai_3] -> Add188/3
  [yita_pesai_3] -> Add182/1
  Product181/1 -> Integrator33/1
  [v1] -> Divide63/1
  Add196/1 -> [e_pesai_3], Scope327/1, Derivative9/1
  [xi_l_dot_3] -> Product142/1
  Add176/1 -> Product161/2
  Divide47/1 -> Subtract23/4
  Divide52/1 -> Subtract28/4
  [k_yita_l_3] -> Product159/1  "k_yita_l"
  Add232/1 -> Product195/1
  [pesai_3] -> Trigonometric Function60/1
  [c_d_pesai_3] -> Gain51/1  "自适应参数"
  [rou_0_3] -> Add226/1
  [v3] -> Divide59/1
  Add182/1 -> Scope274/1, Product24/2
  [yita_l_3] -> Math Function47/1
  Trigonometric Function59/1 -> Product48/2
  [h] -> MATLAB Function23/7(h)
  [fai_3] -> Trigonometric Function65/1
  [xiajie_yuzhi_3] -> Add229/2
  Square3/1 -> [l_ni2_3], Scope238/1
  [v3] -> Divide50/1
  Add157/1 -> Gain49/1
  Derivative53/1 -> Scope284/1
  Product153/1 -> Add183/4
  [h] -> Divide48/1
  [c3_pesai_3] -> Product149/1
  Gain50/1 -> Add151/3
  Memory39/1 -> MATLAB Function38/6(d1b)
  [oumiga_L_dot_1] -> Divide51/3
  [theta_3] -> Trigonometric Function55/1
  ? -> ?
  Derivative66/1 -> Scope421/1
  [pesai_fin_b1_3] -> Memory36/1
  [k_yita_pesai_3] -> Product146/1  "k_yita_pesai"
  [c3_l_3] -> Product166/1
  Add163/1 -> Scope267/1, Product146/3
  Add185/1 -> [shangjie], Scope312/1, MATLAB Function8/2(shangjie)  "上界"
  Trigonometric Function63/1 -> Divide61/2
  [oumiga_1] -> Product48/1
  Constant3/1 -> Math Function41/2
  Derivative55/1 -> Scope254/1, [yipuxilong_pesai_dot_3]
  [yita_l_3] -> Product159/2
  [l_ni2_3] -> Divide57/2
  Derivative47/1 -> Scope321/1
  Product132/1 -> Gain52/1
  Constant67/1 -> Gain47/1
  Integrator41/1 -> Scope280/1
  [v3] -> MATLAB Function22/2(Vi)
  Trigonometric Function64/1 -> Divide56/2
  Add42/1 -> Scope188/1
  Gain30/1 -> [u_21_3]
  [pesai_jie_a1_3] -> Scope405/2, MATLAB Function39/3(jie)
  Add146/1 -> Add42/1, Scope203/1
  [pesai_3] -> Trigonometric Function73/1
  Divide57/1 -> Subtract24/1
  [xi_pesai_0_xia_3_qiehuan] -> MATLAB Function37/1(x0)
  Add158/1 -> Product164/2
  [shang] -> ?
  Constant165/1 -> [k_row_3]
  [c1_l_dot_3] -> Product165/2
  Gain47/1 -> Add175/3
  [fai_3] -> MATLAB Function23/3(fai)
  [pesai_d1_3_dot] -> Add240/1, Scope418/1
  From1046/1 -> Product135/1
  [fai_dot_3] -> Divide48/4
  [pesai_dot_4] -> Gain80/1
  Math Function39/1 -> Product167/1
  [ke_xi_l_3] -> Math Function40/1
  [xi_pesai_0_shang_3_qiehuan] -> Add223/2
  Add150/1 -> [yF3head]
  [fai_dot_3] -> Add197/1
  Product185/1 -> Gain84/1
  [gama_3] -> Add42/2
  [oumiga_1] -> Subtract26/1
  Constant289/1 -> Add227/1
  [yF3head] -> Foolower_3/4(yf1head)
  Math Function41/1 -> Scope318/1, Product23/2
  [k_c_l2_3] -> Product150/1  "k_c_l2"
  Add183/1 -> Product132/1
  Add199/1 -> Product165/1
  [z_l_3] -> Divide54/2
  [c1_pesai_dot_3] -> Product134/2
  [xi_l_3] -> Product142/2
  Add178/1 -> Product157/2
  Product168/1 -> Add181/3
  [yita_pesai_3] -> Add169/1
  Add201/1 -> [xiajie], MATLAB Function8/3(xiajie), Scope313/1
  [z_pesai_3] -> Math Function41/1
  [e_pesai_3] -> Product149/2
  Product24/1 -> Math Function48/1
  [ke_xi_pesai_3] -> Math Function49/1
  [pesai_3] -> Trigonometric Function67/1
  [shangjie_yuzhi_3] -> MATLAB Function36/2(shangjie_yuzhi)
  Derivative9/1 -> [e_pesai_dot_3]
  Constant161/1 -> Math Function42/2
  Gain84/1 -> [yipuxilong_pesai_3], Scope393/1
  [v1] -> Product32/1
  Product192/1 -> Scope392/1, Add224/1
  Product172/1 -> Scope184/1, Add27/1
  [theta_3] -> Subsystem5/11(In11)
  [k_z_pesai_3] -> Product23/1
  Product34/1 -> Abs/1
  Abs/1 -> Add23/1
  Abs1/1 -> Add85/1
  Abs2/1 -> Add69/1
  Abs3/1 -> Add36/1
  Product141/1 -> Abs4/1
  Product169/1 -> Abs5/1
  Abs4/1 -> Scope291/1, Add160/1
  Abs5/1 -> Add186/1
  Constant173/1 -> Add102/1
  Gain64/1 -> Add201/1
  Gain65/1 -> Add201/5
  From1091/1 -> Scope425/2, Switch4/3
  From938/1 -> Gain89/1
  From1112/1 -> Add210/1
  From1092/1 -> MATLAB Function13/1(x0)
  MATLAB Function13/1(shang_) -> Goto572/1, Scope433/1
  From1087/1 -> Scope363/2, Scope373/1, Switch17/1
  Gain88/1 -> Goto559/1, Scope361/1
  From1155/1 -> Add211/1
  Gain89/1 -> Scope374/1, Add211/4
  Add180/1 -> Goto562/1, Scope305/2
  Constant501/1 -> Add208/5
  Switch18/1 -> Switch17/3
  From1154/1 -> Add214/1
  From1108/1 -> Scope352/1, MATLAB Function20/1(d1)
  From1111/1 -> Add210/2
  Add214/1 -> Scope426/1, Scope366/1, Goto564/1
  Add208/1 -> Scope358/1, Scope308/1, Goto567/1
  From1119/1 -> Scope309/2
  Constant502/1 -> Gain87/1
  Constant503/1 -> Add210/5
  Switch17/1 -> Scope363/1, Scope359/1, Goto561/1, Memory15/1, Scope367/1
  From1113/1 -> Add210/4
  Gain87/1 -> Add210/3
  Add213/1 -> Scope432/1, Scope365/1, Goto563/1
  Memory15/1 -> Switch18/1
  MATLAB Function13/2(xia_) -> Goto573/1, Scope434/1
  Constant490/1 -> Goto566/1
  Constant492/1 -> Goto565/1
  From930/1 -> MATLAB Function13/8(xiajie)
  From935/1 -> MATLAB Function13/5(shangjie_yuzhi)
  Gain86/1 -> Add208/3
  From1093/1 -> Scope429/2, Multiport Switch3/4
  From927/1 -> MATLAB Function13/7(shangjie)
  From1152/1 -> Add180/1
  Switch4/1 -> Memory18/1, Scope376/1, Goto560/1, Scope375/1, Scope425/1
  Memory18/1 -> Switch3/1
  From1148/1 -> Add172/4
  Gain95/1 -> Add213/3
  From932/1 -> Memory16/1
  Gain94/1 -> Add214/4, Scope435/1
  From1110/1 -> Add208/4
  From1153/1 -> Add213/1
  From933/1 -> Memory19/1
  From1105/1 -> Add207/4
  Constant497/1 -> Gain85/1
  From1090/1 -> Memory24/1
  Add211/1 -> Goto535/1
  From1101/1 -> Scope365/2, Switch17/2
  From1143/1 -> Product93/1
  From1103/1 -> Add207/2
  Gain92/1 -> Add212/3
  From1089/1 -> Memory23/1
  From1109/1 -> Add208/1
  MATLAB Function13/3(a) -> Scope307/1, Scope431/1, Multiport Switch3/1
  Gain91/1 -> Add211/3
  Memory23/1 -> MATLAB Function13/3(shang)
  Product93/1 -> Gain88/1
  Constant500/1 -> Gain86/1
  Add210/1 -> Scope360/1, Scope309/1, Goto568/1
  Constant491/1 -> Gain96/1, Gain95/1
  Constant495/1 -> Add180/3
  From1114/1 -> Add208/2
  Clock4/1 -> Switch18/2
  MATLAB Function20/1(d) -> Scope304/1, Scope353/1, Goto570/1, Goto569/1
  From959/1 -> Gain90/1
  Memory14/1 -> MATLAB Function20/2(d_)
  Add212/1 -> Goto534/1
  From1118/1 -> Scope308/2
  From1097/1 -> Gain93/1
  Memory16/1 -> MATLAB Function13/9(shangjie_1)
  From1034/1 -> MATLAB Function13/6(xiajie_yuzhi)
  Add167/1 -> Scope305/1
  Clock3/1 -> Switch3/2
  Gain93/1 -> Scope436/1, Add213/4
  From1095/1 -> Scope429/1, Multiport Switch3/3
  Add207/1 -> Scope351/1, MATLAB Function20/4(xiajie)
  From1098/1 -> Gain94/1
  Switch3/1 -> Switch4/1
  From1088/1 -> MATLAB Function13/2(x0_xia)
  From934/1 -> Add212/1
  From1147/1 -> Add172/1
  From1104/1 -> Add207/1
  Multiport Switch3/1 -> Scope430/1, Goto571/1
  Memory24/1 -> MATLAB Function13/4(xia)
  MATLAB Function13/4(shangjie_) -> Goto368/1
  Constant498/1 -> Add207/5
  Memory19/1 -> MATLAB Function13/10(xiajie_1)
  Gain81/1 -> Add172/3
  From1115/1 -> Scope304/3
  Gain85/1 -> Add207/3
  From1150/1 -> Add167/2
  MATLAB Function13/5(xiajie_) -> Goto529/1
  From1146/1 -> Add167/1
  From1151/1 -> Add180/2
  Constant494/1 -> Gain81/1
  From1149/1 -> Memory14/1
  Gain90/1 -> Add212/4, Scope372/1
  From1107/1 -> Scope304/2
  Add172/1 -> Scope350/1, MATLAB Function20/3(shangjie)  "上界"
  MATLAB Function20/2(a) -> Scope307/2
  From1144/1 -> Product93/2
  From1102/1 -> Scope366/2, Switch4/2
  From1094/1 -> Multiport Switch3/2
  Gain96/1 -> Add214/3
  Constant496/1 -> Add172/5
  From1106/1 -> ?
  Constant489/1 -> Gain92/1, Gain91/1
  ? -> Scope362/1
  From1145/1 -> Add172/2
  MATLAB Function49/1(d1) -> [pesai_d1_00_b1]
  [k_tiaota_b1] -> Product94/1
  [xi_pesai_0_xia] -> MATLAB Function48/1(x0)
  Add264/1 -> [pesai_jie_b1], Scope476/1
  Derivative15/1 -> MATLAB Function49/4(d1_dotu)
  [rou_0] -> Gain101/1
  [pesai_jie_b1] -> Scope477/2, MATLAB Function48/3(jie)
  [pesai_d1] -> MATLAB Function49/5(d1_fnu)
  [pesai_d1] -> MATLAB Function49/3(d1u)
  [rou_0] -> Add266/1
  [xiajie_yuzhi] -> MATLAB Function49/2(xiajie_yuzhi)
  Derivative19/1 -> Saturation22/1
  [rou_0] -> Product129/2
  Product95/1 -> Scope472/1, Add264/1
  Product129/1 -> Scope479/1, [xi_pesai_x_b1]
  [xi_pesai_0_xia] -> Add263/1
  [pesai_fin_b1] -> Memory29/1
  Add267/1 -> Gain100/1
  [xi_pesai_x_b1] -> Add267/2
  MATLAB Function48/1(y) -> [pesai_d_b1], Derivative19/1, Scope475/1
  MATLAB Function48/2(a) -> Scope480/1
  [xiajie_yuzhi] -> Add263/2
  [xi_pesai_x_b1] -> Product94/2
  [pesai_fin_b1] -> Scope477/3, MATLAB Function48/4(fin)
  Saturation22/1 -> Scope482/1
  Memory29/1 -> MATLAB Function49/8(d1_fnb)
  [xi_pesai_0_xia] -> MATLAB Function49/1(x0)
  Gain101/1 -> Add265/2
  Memory30/1 -> MATLAB Function49/6(d1b)
  MATLAB Function49/2(d1_dot) -> [pesai_d1_dot_b1]
  MATLAB Function49/3(d1_fn) -> [pesai_fin_b1]
  Constant543/1 -> Add267/1
  [k_tiaota_b1] -> Product110/1
  Product110/1 -> Scope478/1, Add264/2
  Add265/1 -> [k_tiaota_b1]
  [pesai_d1_00_b1] -> Memory30/1
  [pesai_d1] -> Derivative15/1
  [xi_pesai_x_b1] -> Product110/2
  [pesai_d1_dot_b1] -> Add265/1
  [pesai_d1] -> Scope477/1, MATLAB Function48/2(d1)
  Add266/1 -> Product95/1
  Gain100/1 -> Sin3/1
  Product94/1 -> Add266/2
  Memory31/1 -> MATLAB Function49/7(d1_dotb)
  Sin3/1 -> Product95/2
  [pesai_d1_00_b1] -> Scope481/1, Add264/3
  [pesai_d1_dot_b1] -> Memory31/1
  Subtract56/1 -> Product138/2
  Product145/1 -> Subtract60/2
  [theta_3] -> Gain107/1
  [theta_1] -> Subtract71/3
  [xF3head] -> Subtract63/2
  Constant547/1 -> Gain106/1
  [xF1head] -> Subtract66/1
  [xF3head] -> Subtract66/2
  [pesai_1_s] -> Subtract72/3
  Product186/1 -> Scope495/1, [yF1head_s]
  [pesai_1s] -> Trigonometric Function97/1
  [xF3head] -> Subsystem4/2(In2)
  [xF2head] -> Subtract59/1
  [fai_3_s] -> Subtract72/2
  Constant546/1 -> Subtract72/1
  [theta_1] -> Subsystem4/1(In1)
  [xF1head] -> Subsystem4/3(In3)
  Trigonometric Function100/1 -> Product188/1
  [yF1head] -> Subtract62/1
  [yF3head] -> Subtract55/2
  [yF1head] -> Subsystem4/5(In5)
  [yF3head] -> Subtract65/2
  Subtract61/1 -> Trigonometric Function91/1
  Trigonometric Function87/1 -> Product138/1
  [yF1head] -> Subtract65/1
  [yF3head] -> Subsystem4/4(In4)
  [xF1head] -> Subtract63/1
  [yF2head] -> Subtract55/1
  [xF1head_s] -> Scope484/1, Foolower_4/3(x1)
  [yF2head] -> Subtract58/1
  Subtract62/1 -> Product160/1
  Subtract66/1 -> Product183/2
  [xF2head] -> Subtract56/1
  [l_3] -> Product186/2, Product184/2
  [yF1head_s] -> Scope485/1, Foolower_4/4(y1)
  [theta_3] -> Trigonometric Function93/1, Trigonometric Function95/1, Trigonometric Function92/1, Trigonometric Function96/1
  [xF3head] -> Subtract56/2
  Product154/1 -> Subtract60/1
  [theta_3] -> Trigonometric Function94/1, Trigonometric Function90/1, Trigonometric Function89/1, Trigonometric Function87/1
  [yF3head] -> Subtract62/2
  [yF3head] -> Subtract58/2
  [pesai_1_s] -> Subtract67/1
  Subsystem4/1(fai) -> Scope506/1, Subtract39/1
  Product130/1 -> Subtract57/2
  [xF3head] -> Subtract59/2
  Product188/1 -> Scope492/1, [yF2head_s]
  [pesai_2s] -> Trigonometric Function100/1
  [l_4] -> Product188/2, Product187/2
  Foolower_4/1(arc) -> Derivative39/1, Scope504/1, Gain104/1
  Subtract55/1 -> Product130/1
  Subtract67/1 -> Scope490/1, [pesai_1s]
  Trigonometric Function98/1 -> Product186/1
  Product187/1 -> Scope493/1, [xF2head_s]
  Product184/1 -> Scope494/1, [xF1head_s]
  [pesai_2_s] -> Subtract68/1
  Subtract64/1 -> Trigonometric Function91/2
  Product160/1 -> Subtract64/2
  Product171/1 -> Subtract64/1
  Trigonometric Function93/1 -> Product171/1
  Constant534/1 -> Subtract68/2
  Constant544/1 -> Subtract67/2
  [pesai_1s] -> Trigonometric Function98/1
  Trigonometric Function90/1 -> Product145/2
  Trigonometric Function91/1 -> [pesai_1_s], Scope488/1
  Derivative39/1 -> Integrator24/1
  Subtract63/1 -> Product171/2
  Product182/1 -> Subtract61/2
  Subtract68/1 -> Scope491/1, [pesai_2s]
  Product183/1 -> Subtract61/1
  Trigonometric Function97/1 -> Product184/1
  Trigonometric Function99/1 -> Product187/1
  Subtract57/1 -> Trigonometric Function88/2
  Subtract65/1 -> Product182/1
  Subtract60/1 -> Trigonometric Function88/1
  Trigonometric Function96/1 -> Product183/1
  Trigonometric Function92/1 -> Product182/2
  Subtract58/1 -> Product145/1
  Subtract59/1 -> Product154/2
  [xF2head_s] -> Scope507/1, Foolower_4/1(x2)
  Product138/1 -> Subtract57/1
  Trigonometric Function94/1 -> Product154/1
  Trigonometric Function50/1 -> Foolower_4/6(c1)
  Trigonometric Function88/1 -> [pesai_2_s], Scope489/1
  [yF2head_s] -> Scope483/1, Foolower_4/2(y2)
  Foolower_4/2(u2) -> Scope469/1
  Subtract72/1 -> [theta_j0], Scope486/1, Trigonometric Function50/1, Trigonometric Function82/1
  Trigonometric Function82/1 -> Foolower_4/7(s1)
  Integrator24/1 -> Foolower_4/5(u1)
  Trigonometric Function89/1 -> Product130/2
  Trigonometric Function95/1 -> Product160/2
  [pesai_2s] -> Trigonometric Function99/1
  [theta_j0] -> Subtract31/1
  [pesai_2_s] -> Subtract31/2
  Subtract31/1 -> Trigonometric Function103/1
  Trigonometric Function103/1 -> Product189/1
  Product189/1 -> Subtract32/1
  Product190/1 -> Subtract32/2
  [theta_j0] -> Subtract33/1
  Subtract33/1 -> Trigonometric Function104/1
  [pesai_1_s] -> Subtract33/2
  Trigonometric Function104/1 -> Product190/1
  Subtract32/1 -> [wei]
  Subtract34/1 -> Trigonometric Function105/1
  Product205/1 -> Subtract35/2
  [pesai_1_s] -> Subtract36/2
  Product202/1 -> Subtract35/1
  Trigonometric Function106/1 -> Product205/1
  [l_4] -> Product202/2, Product189/2
  [theta_j0] -> Subtract36/1
  [l_3] -> Product205/2, Product190/2
  [theta_j0] -> Subtract34/1
  [pesai_2_s] -> Subtract34/2
  Trigonometric Function105/1 -> Product202/1
  Subtract36/1 -> Trigonometric Function106/1
  Subtract35/1 -> Gain102/1
  [you] -> MATLAB Function50/2("y "), Atan/2
  [wei] -> MATLAB Function50/1(x), Atan/1
  Gain102/1 -> [you]
  Atan/1 -> Scope427/1, [C_3]
  MATLAB Function50/1(y) -> Scope508/1
  [C_3] -> Add102/2
  Subtract40/1 -> Goto584/1, Scope427/2
  [fai_3_s] -> Subtract37/2
  [pesai_1_s] -> Subtract37/3
  Constant551/1 -> Subtract37/1
  Gain107/1 -> Subtract71/2
  [pesai_4] -> Scope489/2
  [pesai_3] -> Scope488/2
  Constant562/1 -> Subtract38/4
  [theta_1] -> Subtract38/3
  [theta_3] -> Subtract38/2
  [pesai_3] -> Subtract38/1
  Constant545/1 -> Subtract39/2
  Subtract39/1 -> [fai_3_s], Scope505/1, Scope518/1
  Subtract38/1 -> Scope505/2, Scope516/1
  Gain104/1 -> Subtract40/1
  Gain106/1 -> Subtract40/2
  Constant563/1 -> Subtract71/1
  [yF2head] -> Foolower_5/2(yl)
  [yF3head] -> Foolower_5/4(yf1head)
  Foolower_5/1(ldot) -> [l_4], Scope519/1
  [xF2head] -> Foolower_5/1(xl)
  [xF3head] -> Foolower_5/3(xf1head)
  Demux/8 -> [k_c_l], [k_c_l_3], [k_c_l_2]
  Demux/2 -> [k_ke_xi_pesai_3], [k_ke_xi_pesai_2], [k_ke_xi_pesai]
  Demux/9 -> [k_c_l2_3], [k_c_l2_2], [k_c_l2]
  Demux/4 -> [k_c_pesai2], [k_c_pesai2_3], [k_c_pesai2_2]
  Demux/6 -> [k_yita_l_3], [k_yita_l_2], [k_yita_l]
  Demux/1 -> [k_yita_pesai], [k_yita_pesai_3], [k_yita_pesai_2]
  Demux/10 -> [k_z_l_3], [k_z_l_2], [k_z_l]
  Mux/1 -> Multiport Switch4/2
  Constant573/1 -> Mux/10
  Constant572/1 -> Mux/9
  Constant570/1 -> Mux/8
  Constant43/1 -> Mux/6
  Demux/7 -> [k_ke_xi_l_3], [k_ke_xi_l_2], [k_ke_xi_l]
  Constant93/1 -> Mux1/4
  Constant106/1 -> Mux1/8
  Demux/3 -> [k_c_pesai_3], [k_c_pesai_2], [k_c_pesai]  "小点好"
  Multiport Switch4/1 -> Demux/1
  Constant36/1 -> Multiport Switch4/1
  Constant567/1 -> Mux/4
  Constant90/1 -> Mux1/10
  Constant568/1 -> Mux/3
  Constant564/1 -> Mux/1
  Demux/5 -> [k_z_pesai_2], [k_z_pesai_3], [k_z_pesai]
  Constant94/1 -> Mux1/3
  Mux2/1 -> Multiport Switch4/4
  Mux1/1 -> Multiport Switch4/3
  Constant105/1 -> Mux1/7
  Constant565/1 -> Mux/5
  Constant101/1 -> Mux1/1
  Constant74/1 -> Mux1/6
  Constant84/1 -> Mux1/9
  Constant14/1 -> Mux2/2
  Constant29/1 -> Mux2/3
  Constant7/1 -> Mux2/6
  Constant109/1 -> Mux1/5
  Constant10/1 -> Mux2/10
  Constant15/1 -> Mux2/4
  Constant32/1 -> Mux2/8
  Constant30/1 -> Mux2/7
  Constant8/1 -> Mux2/1
  Constant33/1 -> Mux2/9
  Constant569/1 -> Mux/7
  Constant9/1 -> Mux2/5
  Constant538/1 -> Mux1/2
  Constant566/1 -> Mux/2
  [rou_0_3] -> MATLAB Function37/6(rou)
  [rou_0_3] -> MATLAB Function38/9(rou)
  [rou_0_3] -> MATLAB Function39/6(rou)
  [rou_0_3] -> MATLAB Function36/9(rou)
  [shangjie_yuzhi] -> MATLAB Function1/5(shangjieyuzhi)
  [rou_0] -> MATLAB Function1/6(rou)
  [xiajie_yuzhi] -> MATLAB Function48/5(xiajieyuzhi)
  [rou_0] -> MATLAB Function48/6(rou)
  [rou_0] -> MATLAB Function2/9(rou)
  [rou_0] -> MATLAB Function49/9(rou)
  [rou_0_2] -> MATLAB Function16/6(rou)
  [rou_0_2] -> MATLAB Function17/9(rou)
  [rou_0_2] -> MATLAB Function15/9(rou)
  [rou_0_2] -> MATLAB Function4/6(rou)
  [shangjie_yuzhi_2] -> MATLAB Function4/5(shangjie)
  [xiajie_yuzhi_2] -> MATLAB Function16/5(xiajieyuzhi)
  [rou_0] -> Saturation Dynamic/1
  Constant38/1 -> Saturation Dynamic/3
  Constant6/1 -> Saturation Dynamic1/3
  [rou_0] -> Saturation Dynamic1/1
  Add263/1 -> Saturation Dynamic1/2
  Saturation Dynamic1/1 -> Product129/1
  Constant12/1 -> Saturation Dynamic2/3
  [rou_0_2] -> Saturation Dynamic2/1
  Add134/1 -> Saturation Dynamic2/2
  Saturation Dynamic2/1 -> Product126/1
  Saturation Dynamic3/1 -> Product128/1
  Add139/1 -> Saturation Dynamic3/2
  Constant13/1 -> Saturation Dynamic3/3
  [rou_0_2] -> Saturation Dynamic3/1
  Saturation Dynamic4/1 -> Product198/1
  Add229/1 -> Saturation Dynamic4/2
  Constant39/1 -> Saturation Dynamic4/3
  [rou_0_3] -> Saturation Dynamic4/1
  Saturation Dynamic5/1 -> Product196/1
  Add223/1 -> Saturation Dynamic5/2
  Constant41/1 -> Saturation Dynamic5/3
  [rou_0_3] -> Saturation Dynamic5/1
  Constant5/1 -> [rou_0_2]
  Constant152/1 -> [shangjie_yuzhi_2]  "数据值不能改， 涉及到右边的数据计算"
  Constant122/1 -> [xiajie_yuzhi_2]
  Constant11/1 -> [rou_0]
  Constant88/1 -> [shangjie_yuzhi]
  Constant52/1 -> [xiajie_yuzhi]
  Constant4/1 -> [rou_0_3]
  Constant243/1 -> [xiajie_yuzhi_3]
  Constant247/1 -> [shangjie_yuzhi_3]
  [chushi_3] -> Integrator45/2
  [chushi_1] -> Integrator9/2
  [chushi_2] -> Integrator30/2
  [chushi] -> Integrator11/2
  Demux1/2 -> [chushi_1]
  Demux1/3 -> [chushi_2]
  Demux1/4 -> [chushi_3]
  Demux1/1 -> [chushi]
  Gain25/1 -> Product33/2
  Constant107/1 -> Mux3/8
  Constant91/1 -> Mux3/4
  Constant104/1 -> Mux3/7
  Constant73/1 -> Mux3/6
  Constant111/1 -> Mux3/9
  Constant92/1 -> Mux3/3
  Constant86/1 -> Mux3/2
  Constant78/1 -> Mux3/1
  Constant113/1 -> Mux3/10
  Constant85/1 -> Mux3/5
  Mux3/1 -> Multiport Switch4/5
  Mux6/1 -> Multiport Switch4/6
  Constant176/1 -> Mux6/1
  Constant157/1 -> Mux6/10
  Constant166/1 -> Mux6/6
  Constant182/1 -> Mux6/2
  Constant156/1 -> Mux6/9
  Constant186/1 -> Mux6/3
  Constant150/1 -> Mux6/7
  Constant178/1 -> Mux6/5
  Constant154/1 -> Mux6/8
  Constant185/1 -> Mux6/4
  Constant190/1 -> Mux7/3
  Constant194/1 -> Mux7/1
  Constant193/1 -> Mux7/4
  Constant187/1 -> Mux7/2
  Constant195/1 -> [r]
  Constant202/1 -> [Iz]
  Constant196/1 -> [m]
  Constant203/1 -> [zhouju]
  [v1_dot_liju] -> MATLAB Function32/5(v_dot)
  [oumiga_1_dot_liju] -> MATLAB Function32/6(oumiga_dot)
  [Iz] -> MATLAB Function32/4(Iz)
  [m] -> MATLAB Function32/3(m)
  [r] -> MATLAB Function32/2(r)
  [zhouju] -> MATLAB Function32/1(zhouju)
  MATLAB Function32/1(t1) -> [t1_1], Scope36/1, Scope34/1
  MATLAB Function32/2(t2) -> [t2_1], Scope36/2, Scope35/1
  [r] -> MATLAB Function47/2(r)
  MATLAB Function47/1(t1) -> Scope41/1, [t1_2], Scope37/1
  [zhouju] -> MATLAB Function47/1(zhouju)
  MATLAB Function47/2(t2) -> Scope41/2, [t2_2], Scope39/1
  [m] -> MATLAB Function47/3(m)
  [oumiga_2_dot_liju] -> MATLAB Function47/6(oumiga_dot)
  [v2_dot_liju] -> MATLAB Function47/5(v_dot)
  [Iz] -> MATLAB Function47/4(Iz)
  MATLAB Function52/2(t2) -> Scope289/2, [t2_3], Scope286/1
  [m] -> MATLAB Function52/3(m)
  [Iz] -> MATLAB Function52/4(Iz)
  [oumiga_3_dot_liju] -> MATLAB Function52/6(oumiga_dot)
  [v3_dot_liju] -> MATLAB Function52/5(v_dot)
  MATLAB Function52/1(t1) -> Scope289/1, [t1_3], Scope44/1
  [r] -> MATLAB Function52/2(r)
  [zhouju] -> MATLAB Function52/1(zhouju)
  Gain66/1 -> [xi_l_xia]
  Gain68/1 -> [xi_l_2_xia]
  Gain69/1 -> [xi_l_3_xia]
  Constant217/1 -> Mux15/5
  Constant220/1 -> Mux15/3
  Mux15/1 -> Multiport Switch4/7
  Constant218/1 -> Mux15/2
  Constant213/1 -> Mux15/9
  Constant212/1 -> Mux15/8
  Constant219/1 -> Mux15/4
  Constant211/1 -> Mux15/7
  Constant215/1 -> Mux15/6
  Constant216/1 -> Mux15/1
  Constant214/1 -> Mux15/10
  Derivative/1 -> [l_dot_3]
  [l_3] -> Derivative/1
  [pesai_3] -> Derivative3/1
  Derivative3/1 -> [pesai_dot_3]
  [l_2] -> Derivative4/1
  Derivative4/1 -> [l_dot_2]
  [pesai_2] -> Derivative24/1
  Derivative24/1 -> [pesai_dot_2]
  [l] -> Derivative51/1
  Derivative51/1 -> [l_dot]
  [pesai] -> Derivative58/1
  Derivative58/1 -> [pesai_dot]
  Mux7/1 -> Demux1/1
  Gain83/1 -> [oumiga_L], Scope30/1
  Add270/1 -> MATLAB 需要跑30s6/2(t)
  Constant31/1 -> [vL]  "<X>"
  MATLAB 需要跑30s6/1(y) -> Gain83/1
  Clock24/1 -> Add270/1
